simulink model "model"  (R2016a)
(part 3 of 5)

  _CN_258020275_275000_CN_178983951_275000 : powerlib/Elements/Distributed Parameters Line  Phases=3  Frequency=50  Resistance=[0.01273 0.3864]  Inductance="[0.9337e-3  4.1264e-3]"  Capacitance=[12.74e-9 7.751e-9]  Length=72.4946  x1=[8.73114913702011e-11 380000 380000;314.159265358979 314.159265358979 314.159265358979;-0.177670123217348 0.415246442777429 -1.15554988401747]  x2=[1.26090477118469e-09 381852.398472139 381852.398472139;314.159265358979 314.159265358979 314.159265358979;-1.41941675517191 0.415007521738739 -1.15578880505616]  x3=[1.07663708898761e-11 1405.24743813465 1405.24743813466;314.159265358979 314.159265358979 314.159265358979;-2.70558821102223 0.316110507002444 -1.25468581979246]  x4=[8.62234243168895e-12 1405.96374414071 1405.9637441407;314.159265358979 314.159265358979 314.159265358979;0.245769282942371 0.405640215255436 -1.16515611153945]  x5=0.000565541566995742  V1=ones(3,3)  V2=ones(3,3)  I1=ones(3,3)  I2=ones(3,3)  nHarmo=1  Measurements=None
  _CN_258020275_275000_CN_184552955_275000 : powerlib/Elements/Distributed Parameters Line  Phases=3  Frequency=50  Resistance=[0.01273 0.3864]  Inductance="[0.9337e-3  4.1264e-3]"  Capacitance=[12.74e-9 7.751e-9]  Length=80.3266  x1=[8.73114913702011e-11 380000 380000;314.159265358979 314.159265358979 314.159265358979;-0.177670123217348 0.415246442777429 -1.15554988401747]  x2=[1.26090477118469e-09 381852.398472139 381852.398472139;314.159265358979 314.159265358979 314.159265358979;-1.41941675517191 0.415007521738739 -1.15578880505616]  x3=[1.07663708898761e-11 1405.24743813465 1405.24743813466;314.159265358979 314.159265358979 314.159265358979;-2.70558821102223 0.316110507002444 -1.25468581979246]  x4=[8.62234243168895e-12 1405.96374414071 1405.9637441407;314.159265358979 314.159265358979 314.159265358979;0.245769282942371 0.405640215255436 -1.16515611153945]  x5=0.000565541566995742  V1=ones(3,3)  V2=ones(3,3)  I1=ones(3,3)  I2=ones(3,3)  nHarmo=1  Measurements=None
  _CN_262495875_132000_CN_185153858_132000 : powerlib/Elements/Distributed Parameters Line  Phases=3  Frequency=50  Resistance=[0.01273 0.3864]  Inductance="[0.9337e-3  4.1264e-3]"  Capacitance=[12.74e-9 7.751e-9]  Length=25.9236  x1=[8.73114913702011e-11 380000 380000;314.159265358979 314.159265358979 314.159265358979;-0.177670123217348 0.415246442777429 -1.15554988401747]  x2=[1.26090477118469e-09 381852.398472139 381852.398472139;314.159265358979 314.159265358979 314.159265358979;-1.41941675517191 0.415007521738739 -1.15578880505616]  x3=[1.07663708898761e-11 1405.24743813465 1405.24743813466;314.159265358979 314.159265358979 314.159265358979;-2.70558821102223 0.316110507002444 -1.25468581979246]  x4=[8.62234243168895e-12 1405.96374414071 1405.9637441407;314.159265358979 314.159265358979 314.159265358979;0.245769282942371 0.405640215255436 -1.16515611153945]  x5=0.000565541566995742  V1=ones(3,3)  V2=ones(3,3)  I1=ones(3,3)  I2=ones(3,3)  nHarmo=1  Measurements=None
  _CN_28088740_275000_CN_42209860_275000 : powerlib/Elements/Distributed Parameters Line  Phases=3  Frequency=50  Resistance=[0.01273 0.3864]  Inductance="[0.9337e-3  4.1264e-3]"  Capacitance=[12.74e-9 7.751e-9]  Length=14.7594  x1=[8.73114913702011e-11 380000 380000;314.159265358979 314.159265358979 314.159265358979;-0.177670123217348 0.415246442777429 -1.15554988401747]  x2=[1.26090477118469e-09 381852.398472139 381852.398472139;314.159265358979 314.159265358979 314.159265358979;-1.41941675517191 0.415007521738739 -1.15578880505616]  x3=[1.07663708898761e-11 1405.24743813465 1405.24743813466;314.159265358979 314.159265358979 314.159265358979;-2.70558821102223 0.316110507002444 -1.25468581979246]  x4=[8.62234243168895e-12 1405.96374414071 1405.9637441407;314.159265358979 314.159265358979 314.159265358979;0.245769282942371 0.405640215255436 -1.16515611153945]  x5=0.000565541566995742  V1=ones(3,3)  V2=ones(3,3)  I1=ones(3,3)  I2=ones(3,3)  nHarmo=1  Measurements=None
  _CN_28088740_275000_CN_83525879_275000 : powerlib/Elements/Distributed Parameters Line  Phases=3  Frequency=50  Resistance=[0.01273 0.3864]  Inductance="[0.9337e-3  4.1264e-3]"  Capacitance=[12.74e-9 7.751e-9]  Length=33.294  x1=[8.73114913702011e-11 380000 380000;314.159265358979 314.159265358979 314.159265358979;-0.177670123217348 0.415246442777429 -1.15554988401747]  x2=[1.26090477118469e-09 381852.398472139 381852.398472139;314.159265358979 314.159265358979 314.159265358979;-1.41941675517191 0.415007521738739 -1.15578880505616]  x3=[1.07663708898761e-11 1405.24743813465 1405.24743813466;314.159265358979 314.159265358979 314.159265358979;-2.70558821102223 0.316110507002444 -1.25468581979246]  x4=[8.62234243168895e-12 1405.96374414071 1405.9637441407;314.159265358979 314.159265358979 314.159265358979;0.245769282942371 0.405640215255436 -1.16515611153945]  x5=0.000565541566995742  V1=ones(3,3)  V2=ones(3,3)  I1=ones(3,3)  I2=ones(3,3)  nHarmo=1  Measurements=None
  _CN_337464444_132000_CN_337464445_132000 : powerlib/Elements/Distributed Parameters Line  Phases=3  Frequency=50  Resistance=[0.01273 0.3864]  Inductance="[0.9337e-3  4.1264e-3]"  Capacitance=[12.74e-9 7.751e-9]  Length=37.3019  x1=[8.73114913702011e-11 380000 380000;314.159265358979 314.159265358979 314.159265358979;-0.177670123217348 0.415246442777429 -1.15554988401747]  x2=[1.26090477118469e-09 381852.398472139 381852.398472139;314.159265358979 314.159265358979 314.159265358979;-1.41941675517191 0.415007521738739 -1.15578880505616]  x3=[1.07663708898761e-11 1405.24743813465 1405.24743813466;314.159265358979 314.159265358979 314.159265358979;-2.70558821102223 0.316110507002444 -1.25468581979246]  x4=[8.62234243168895e-12 1405.96374414071 1405.9637441407;314.159265358979 314.159265358979 314.159265358979;0.245769282942371 0.405640215255436 -1.16515611153945]  x5=0.000565541566995742  V1=ones(3,3)  V2=ones(3,3)  I1=ones(3,3)  I2=ones(3,3)  nHarmo=1  Measurements=None
  _CN_337464445_132000_CN_120941257_132000 : powerlib/Elements/Distributed Parameters Line  Phases=3  Frequency=50  Resistance=[0.01273 0.3864]  Inductance="[0.9337e-3  4.1264e-3]"  Capacitance=[12.74e-9 7.751e-9]  Length=17.2696  x1=[8.73114913702011e-11 380000 380000;314.159265358979 314.159265358979 314.159265358979;-0.177670123217348 0.415246442777429 -1.15554988401747]  x2=[1.26090477118469e-09 381852.398472139 381852.398472139;314.159265358979 314.159265358979 314.159265358979;-1.41941675517191 0.415007521738739 -1.15578880505616]  x3=[1.07663708898761e-11 1405.24743813465 1405.24743813466;314.159265358979 314.159265358979 314.159265358979;-2.70558821102223 0.316110507002444 -1.25468581979246]  x4=[8.62234243168895e-12 1405.96374414071 1405.9637441407;314.159265358979 314.159265358979 314.159265358979;0.245769282942371 0.405640215255436 -1.16515611153945]  x5=0.000565541566995742  V1=ones(3,3)  V2=ones(3,3)  I1=ones(3,3)  I2=ones(3,3)  nHarmo=1  Measurements=None
  _CN_363326105_275000_CN_179856840_275000 : powerlib/Elements/Distributed Parameters Line  Phases=3  Frequency=50  Resistance=[0.01273 0.3864]  Inductance="[0.9337e-3  4.1264e-3]"  Capacitance=[12.74e-9 7.751e-9]  Length=82.6904  x1=[8.73114913702011e-11 380000 380000;314.159265358979 314.159265358979 314.159265358979;-0.177670123217348 0.415246442777429 -1.15554988401747]  x2=[1.26090477118469e-09 381852.398472139 381852.398472139;314.159265358979 314.159265358979 314.159265358979;-1.41941675517191 0.415007521738739 -1.15578880505616]  x3=[1.07663708898761e-11 1405.24743813465 1405.24743813466;314.159265358979 314.159265358979 314.159265358979;-2.70558821102223 0.316110507002444 -1.25468581979246]  x4=[8.62234243168895e-12 1405.96374414071 1405.9637441407;314.159265358979 314.159265358979 314.159265358979;0.245769282942371 0.405640215255436 -1.16515611153945]  x5=0.000565541566995742  V1=ones(3,3)  V2=ones(3,3)  I1=ones(3,3)  I2=ones(3,3)  nHarmo=1  Measurements=None
  _CN_386388564_400000_CN_418832515_400000 : powerlib/Elements/Distributed Parameters Line  Phases=3  Frequency=50  Resistance=[0.01273 0.3864]  Inductance="[0.9337e-3  4.1264e-3]"  Capacitance=[12.74e-9 7.751e-9]  Length=233.4949  x1=[8.73114913702011e-11 380000 380000;314.159265358979 314.159265358979 314.159265358979;-0.177670123217348 0.415246442777429 -1.15554988401747]  x2=[1.26090477118469e-09 381852.398472139 381852.398472139;314.159265358979 314.159265358979 314.159265358979;-1.41941675517191 0.415007521738739 -1.15578880505616]  x3=[1.07663708898761e-11 1405.24743813465 1405.24743813466;314.159265358979 314.159265358979 314.159265358979;-2.70558821102223 0.316110507002444 -1.25468581979246]  x4=[8.62234243168895e-12 1405.96374414071 1405.9637441407;314.159265358979 314.159265358979 314.159265358979;0.245769282942371 0.405640215255436 -1.16515611153945]  x5=0.000565541566995742  V1=ones(3,3)  V2=ones(3,3)  I1=ones(3,3)  I2=ones(3,3)  nHarmo=1  Measurements=None
  _CN_42209493_132000_CN_81813288_132000 : powerlib/Elements/Distributed Parameters Line  Phases=3  Frequency=50  Resistance=[0.01273 0.3864]  Inductance="[0.9337e-3  4.1264e-3]"  Capacitance=[12.74e-9 7.751e-9]  Length=3.3802  x1=[8.73114913702011e-11 380000 380000;314.159265358979 314.159265358979 314.159265358979;-0.177670123217348 0.415246442777429 -1.15554988401747]  x2=[1.26090477118469e-09 381852.398472139 381852.398472139;314.159265358979 314.159265358979 314.159265358979;-1.41941675517191 0.415007521738739 -1.15578880505616]  x3=[1.07663708898761e-11 1405.24743813465 1405.24743813466;314.159265358979 314.159265358979 314.159265358979;-2.70558821102223 0.316110507002444 -1.25468581979246]  x4=[8.62234243168895e-12 1405.96374414071 1405.9637441407;314.159265358979 314.159265358979 314.159265358979;0.245769282942371 0.405640215255436 -1.16515611153945]  x5=0.000565541566995742  V1=ones(3,3)  V2=ones(3,3)  I1=ones(3,3)  I2=ones(3,3)  nHarmo=1  Measurements=None
  _CN_42209493_275000_CN_81817181_275000 : powerlib/Elements/Distributed Parameters Line  Phases=3  Frequency=50  Resistance=[0.01273 0.3864]  Inductance="[0.9337e-3  4.1264e-3]"  Capacitance=[12.74e-9 7.751e-9]  Length=11.3863  x1=[8.73114913702011e-11 380000 380000;314.159265358979 314.159265358979 314.159265358979;-0.177670123217348 0.415246442777429 -1.15554988401747]  x2=[1.26090477118469e-09 381852.398472139 381852.398472139;314.159265358979 314.159265358979 314.159265358979;-1.41941675517191 0.415007521738739 -1.15578880505616]  x3=[1.07663708898761e-11 1405.24743813465 1405.24743813466;314.159265358979 314.159265358979 314.159265358979;-2.70558821102223 0.316110507002444 -1.25468581979246]  x4=[8.62234243168895e-12 1405.96374414071 1405.9637441407;314.159265358979 314.159265358979 314.159265358979;0.245769282942371 0.405640215255436 -1.16515611153945]  x5=0.000565541566995742  V1=ones(3,3)  V2=ones(3,3)  I1=ones(3,3)  I2=ones(3,3)  nHarmo=1  Measurements=None
  _CN_42209860_275000_CN_178944143_275000 : powerlib/Elements/Distributed Parameters Line  Phases=3  Frequency=50  Resistance=[0.01273 0.3864]  Inductance="[0.9337e-3  4.1264e-3]"  Capacitance=[12.74e-9 7.751e-9]  Length=11.1612  x1=[8.73114913702011e-11 380000 380000;314.159265358979 314.159265358979 314.159265358979;-0.177670123217348 0.415246442777429 -1.15554988401747]  x2=[1.26090477118469e-09 381852.398472139 381852.398472139;314.159265358979 314.159265358979 314.159265358979;-1.41941675517191 0.415007521738739 -1.15578880505616]  x3=[1.07663708898761e-11 1405.24743813465 1405.24743813466;314.159265358979 314.159265358979 314.159265358979;-2.70558821102223 0.316110507002444 -1.25468581979246]  x4=[8.62234243168895e-12 1405.96374414071 1405.9637441407;314.159265358979 314.159265358979 314.159265358979;0.245769282942371 0.405640215255436 -1.16515611153945]  x5=0.000565541566995742  V1=ones(3,3)  V2=ones(3,3)  I1=ones(3,3)  I2=ones(3,3)  nHarmo=1  Measurements=None
  _CN_42209860_275000_CN_42209493_275000 : powerlib/Elements/Distributed Parameters Line  Phases=3  Frequency=50  Resistance=[0.01273 0.3864]  Inductance="[0.9337e-3  4.1264e-3]"  Capacitance=[12.74e-9 7.751e-9]  Length=2.13  x1=[8.73114913702011e-11 380000 380000;314.159265358979 314.159265358979 314.159265358979;-0.177670123217348 0.415246442777429 -1.15554988401747]  x2=[1.26090477118469e-09 381852.398472139 381852.398472139;314.159265358979 314.159265358979 314.159265358979;-1.41941675517191 0.415007521738739 -1.15578880505616]  x3=[1.07663708898761e-11 1405.24743813465 1405.24743813466;314.159265358979 314.159265358979 314.159265358979;-2.70558821102223 0.316110507002444 -1.25468581979246]  x4=[8.62234243168895e-12 1405.96374414071 1405.9637441407;314.159265358979 314.159265358979 314.159265358979;0.245769282942371 0.405640215255436 -1.16515611153945]  x5=0.000565541566995742  V1=ones(3,3)  V2=ones(3,3)  I1=ones(3,3)  I2=ones(3,3)  nHarmo=1  Measurements=None
  _CN_59037450_132000_CN_62191005_132000 : powerlib/Elements/Distributed Parameters Line  Phases=3  Frequency=50  Resistance=[0.01273 0.3864]  Inductance="[0.9337e-3  4.1264e-3]"  Capacitance=[12.74e-9 7.751e-9]  Length=22.8456  x1=[8.73114913702011e-11 380000 380000;314.159265358979 314.159265358979 314.159265358979;-0.177670123217348 0.415246442777429 -1.15554988401747]  x2=[1.26090477118469e-09 381852.398472139 381852.398472139;314.159265358979 314.159265358979 314.159265358979;-1.41941675517191 0.415007521738739 -1.15578880505616]  x3=[1.07663708898761e-11 1405.24743813465 1405.24743813466;314.159265358979 314.159265358979 314.159265358979;-2.70558821102223 0.316110507002444 -1.25468581979246]  x4=[8.62234243168895e-12 1405.96374414071 1405.9637441407;314.159265358979 314.159265358979 314.159265358979;0.245769282942371 0.405640215255436 -1.16515611153945]  x5=0.000565541566995742  V1=ones(3,3)  V2=ones(3,3)  I1=ones(3,3)  I2=ones(3,3)  nHarmo=1  Measurements=None
  _CN_59037450_132000_CN_62208493_132000 : powerlib/Elements/Distributed Parameters Line  Phases=3  Frequency=50  Resistance=[0.01273 0.3864]  Inductance="[0.9337e-3  4.1264e-3]"  Capacitance=[12.74e-9 7.751e-9]  Length=4.1197  x1=[8.73114913702011e-11 380000 380000;314.159265358979 314.159265358979 314.159265358979;-0.177670123217348 0.415246442777429 -1.15554988401747]  x2=[1.26090477118469e-09 381852.398472139 381852.398472139;314.159265358979 314.159265358979 314.159265358979;-1.41941675517191 0.415007521738739 -1.15578880505616]  x3=[1.07663708898761e-11 1405.24743813465 1405.24743813466;314.159265358979 314.159265358979 314.159265358979;-2.70558821102223 0.316110507002444 -1.25468581979246]  x4=[8.62234243168895e-12 1405.96374414071 1405.9637441407;314.159265358979 314.159265358979 314.159265358979;0.245769282942371 0.405640215255436 -1.16515611153945]  x5=0.000565541566995742  V1=ones(3,3)  V2=ones(3,3)  I1=ones(3,3)  I2=ones(3,3)  nHarmo=1  Measurements=None
  _CN_62191005_400000_CN_120584910_400000 : powerlib/Elements/Distributed Parameters Line  Phases=3  Frequency=50  Resistance=[0.01273 0.3864]  Inductance="[0.9337e-3  4.1264e-3]"  Capacitance=[12.74e-9 7.751e-9]  Length=16.2899  x1=[8.73114913702011e-11 380000 380000;314.159265358979 314.159265358979 314.159265358979;-0.177670123217348 0.415246442777429 -1.15554988401747]  x2=[1.26090477118469e-09 381852.398472139 381852.398472139;314.159265358979 314.159265358979 314.159265358979;-1.41941675517191 0.415007521738739 -1.15578880505616]  x3=[1.07663708898761e-11 1405.24743813465 1405.24743813466;314.159265358979 314.159265358979 314.159265358979;-2.70558821102223 0.316110507002444 -1.25468581979246]  x4=[8.62234243168895e-12 1405.96374414071 1405.9637441407;314.159265358979 314.159265358979 314.159265358979;0.245769282942371 0.405640215255436 -1.16515611153945]  x5=0.000565541566995742  V1=ones(3,3)  V2=ones(3,3)  I1=ones(3,3)  I2=ones(3,3)  nHarmo=1  Measurements=None
  _CN_62191005_400000_CN_177800991_400000 : powerlib/Elements/Distributed Parameters Line  Phases=3  Frequency=50  Resistance=[0.01273 0.3864]  Inductance="[0.9337e-3  4.1264e-3]"  Capacitance=[12.74e-9 7.751e-9]  Length=108.9818  x1=[8.73114913702011e-11 380000 380000;314.159265358979 314.159265358979 314.159265358979;-0.177670123217348 0.415246442777429 -1.15554988401747]  x2=[1.26090477118469e-09 381852.398472139 381852.398472139;314.159265358979 314.159265358979 314.159265358979;-1.41941675517191 0.415007521738739 -1.15578880505616]  x3=[1.07663708898761e-11 1405.24743813465 1405.24743813466;314.159265358979 314.159265358979 314.159265358979;-2.70558821102223 0.316110507002444 -1.25468581979246]  x4=[8.62234243168895e-12 1405.96374414071 1405.9637441407;314.159265358979 314.159265358979 314.159265358979;0.245769282942371 0.405640215255436 -1.16515611153945]  x5=0.000565541566995742  V1=ones(3,3)  V2=ones(3,3)  I1=ones(3,3)  I2=ones(3,3)  nHarmo=1  Measurements=None
  _CN_62191005_400000_CN_219384657_400000 : powerlib/Elements/Distributed Parameters Line  Phases=3  Frequency=50  Resistance=[0.01273 0.3864]  Inductance="[0.9337e-3  4.1264e-3]"  Capacitance=[12.74e-9 7.751e-9]  Length=32.1405  x1=[8.73114913702011e-11 380000 380000;314.159265358979 314.159265358979 314.159265358979;-0.177670123217348 0.415246442777429 -1.15554988401747]  x2=[1.26090477118469e-09 381852.398472139 381852.398472139;314.159265358979 314.159265358979 314.159265358979;-1.41941675517191 0.415007521738739 -1.15578880505616]  x3=[1.07663708898761e-11 1405.24743813465 1405.24743813466;314.159265358979 314.159265358979 314.159265358979;-2.70558821102223 0.316110507002444 -1.25468581979246]  x4=[8.62234243168895e-12 1405.96374414071 1405.9637441407;314.159265358979 314.159265358979 314.159265358979;0.245769282942371 0.405640215255436 -1.16515611153945]  x5=0.000565541566995742  V1=ones(3,3)  V2=ones(3,3)  I1=ones(3,3)  I2=ones(3,3)  nHarmo=1  Measurements=None
  _CN_62191005_400000_CN_252396496_132000 : powerlib/Elements/Distributed Parameters Line  Phases=3  Frequency=50  Resistance=[0.01273 0.3864]  Inductance="[0.9337e-3  4.1264e-3]"  Capacitance=[12.74e-9 7.751e-9]  Length=40.4547  x1=[8.73114913702011e-11 380000 380000;314.159265358979 314.159265358979 314.159265358979;-0.177670123217348 0.415246442777429 -1.15554988401747]  x2=[1.26090477118469e-09 381852.398472139 381852.398472139;314.159265358979 314.159265358979 314.159265358979;-1.41941675517191 0.415007521738739 -1.15578880505616]  x3=[1.07663708898761e-11 1405.24743813465 1405.24743813466;314.159265358979 314.159265358979 314.159265358979;-2.70558821102223 0.316110507002444 -1.25468581979246]  x4=[8.62234243168895e-12 1405.96374414071 1405.9637441407;314.159265358979 314.159265358979 314.159265358979;0.245769282942371 0.405640215255436 -1.16515611153945]  x5=0.000565541566995742  V1=ones(3,3)  V2=ones(3,3)  I1=ones(3,3)  I2=ones(3,3)  nHarmo=1  Measurements=None
  _CN_62191005_400000_CN_62193952_400000 : powerlib/Elements/Distributed Parameters Line  Phases=3  Frequency=50  Resistance=[0.01273 0.3864]  Inductance="[0.9337e-3  4.1264e-3]"  Capacitance=[12.74e-9 7.751e-9]  Length=47.199  x1=[8.73114913702011e-11 380000 380000;314.159265358979 314.159265358979 314.159265358979;-0.177670123217348 0.415246442777429 -1.15554988401747]  x2=[1.26090477118469e-09 381852.398472139 381852.398472139;314.159265358979 314.159265358979 314.159265358979;-1.41941675517191 0.415007521738739 -1.15578880505616]  x3=[1.07663708898761e-11 1405.24743813465 1405.24743813466;314.159265358979 314.159265358979 314.159265358979;-2.70558821102223 0.316110507002444 -1.25468581979246]  x4=[8.62234243168895e-12 1405.96374414071 1405.9637441407;314.159265358979 314.159265358979 314.159265358979;0.245769282942371 0.405640215255436 -1.16515611153945]  x5=0.000565541566995742  V1=ones(3,3)  V2=ones(3,3)  I1=ones(3,3)  I2=ones(3,3)  nHarmo=1  Measurements=None
  _CN_62193952_400000_CN_252396496_132000 : powerlib/Elements/Distributed Parameters Line  Phases=3  Frequency=50  Resistance=[0.01273 0.3864]  Inductance="[0.9337e-3  4.1264e-3]"  Capacitance=[12.74e-9 7.751e-9]  Length=31.3538  x1=[8.73114913702011e-11 380000 380000;314.159265358979 314.159265358979 314.159265358979;-0.177670123217348 0.415246442777429 -1.15554988401747]  x2=[1.26090477118469e-09 381852.398472139 381852.398472139;314.159265358979 314.159265358979 314.159265358979;-1.41941675517191 0.415007521738739 -1.15578880505616]  x3=[1.07663708898761e-11 1405.24743813465 1405.24743813466;314.159265358979 314.159265358979 314.159265358979;-2.70558821102223 0.316110507002444 -1.25468581979246]  x4=[8.62234243168895e-12 1405.96374414071 1405.9637441407;314.159265358979 314.159265358979 314.159265358979;0.245769282942371 0.405640215255436 -1.16515611153945]  x5=0.000565541566995742  V1=ones(3,3)  V2=ones(3,3)  I1=ones(3,3)  I2=ones(3,3)  nHarmo=1  Measurements=None
  _CN_62193952_400000_CN_62218063_400000 : powerlib/Elements/Distributed Parameters Line  Phases=3  Frequency=50  Resistance=[0.01273 0.3864]  Inductance="[0.9337e-3  4.1264e-3]"  Capacitance=[12.74e-9 7.751e-9]  Length=12.3981  x1=[8.73114913702011e-11 380000 380000;314.159265358979 314.159265358979 314.159265358979;-0.177670123217348 0.415246442777429 -1.15554988401747]  x2=[1.26090477118469e-09 381852.398472139 381852.398472139;314.159265358979 314.159265358979 314.159265358979;-1.41941675517191 0.415007521738739 -1.15578880505616]  x3=[1.07663708898761e-11 1405.24743813465 1405.24743813466;314.159265358979 314.159265358979 314.159265358979;-2.70558821102223 0.316110507002444 -1.25468581979246]  x4=[8.62234243168895e-12 1405.96374414071 1405.9637441407;314.159265358979 314.159265358979 314.159265358979;0.245769282942371 0.405640215255436 -1.16515611153945]  x5=0.000565541566995742  V1=ones(3,3)  V2=ones(3,3)  I1=ones(3,3)  I2=ones(3,3)  nHarmo=1  Measurements=None
  _CN_62216709_132000_CN_402366747_132000 : powerlib/Elements/Distributed Parameters Line  Phases=3  Frequency=50  Resistance=[0.01273 0.3864]  Inductance="[0.9337e-3  4.1264e-3]"  Capacitance=[12.74e-9 7.751e-9]  Length=1.8763  x1=[8.73114913702011e-11 380000 380000;314.159265358979 314.159265358979 314.159265358979;-0.177670123217348 0.415246442777429 -1.15554988401747]  x2=[1.26090477118469e-09 381852.398472139 381852.398472139;314.159265358979 314.159265358979 314.159265358979;-1.41941675517191 0.415007521738739 -1.15578880505616]  x3=[1.07663708898761e-11 1405.24743813465 1405.24743813466;314.159265358979 314.159265358979 314.159265358979;-2.70558821102223 0.316110507002444 -1.25468581979246]  x4=[8.62234243168895e-12 1405.96374414071 1405.9637441407;314.159265358979 314.159265358979 314.159265358979;0.245769282942371 0.405640215255436 -1.16515611153945]  x5=0.000565541566995742  V1=ones(3,3)  V2=ones(3,3)  I1=ones(3,3)  I2=ones(3,3)  nHarmo=1  Measurements=None
  _CN_62216709_132000_CN_62208493_132000 : powerlib/Elements/Distributed Parameters Line  Phases=3  Frequency=50  Resistance=[0.01273 0.3864]  Inductance="[0.9337e-3  4.1264e-3]"  Capacitance=[12.74e-9 7.751e-9]  Length=6.6911  x1=[8.73114913702011e-11 380000 380000;314.159265358979 314.159265358979 314.159265358979;-0.177670123217348 0.415246442777429 -1.15554988401747]  x2=[1.26090477118469e-09 381852.398472139 381852.398472139;314.159265358979 314.159265358979 314.159265358979;-1.41941675517191 0.415007521738739 -1.15578880505616]  x3=[1.07663708898761e-11 1405.24743813465 1405.24743813466;314.159265358979 314.159265358979 314.159265358979;-2.70558821102223 0.316110507002444 -1.25468581979246]  x4=[8.62234243168895e-12 1405.96374414071 1405.9637441407;314.159265358979 314.159265358979 314.159265358979;0.245769282942371 0.405640215255436 -1.16515611153945]  x5=0.000565541566995742  V1=ones(3,3)  V2=ones(3,3)  I1=ones(3,3)  I2=ones(3,3)  nHarmo=1  Measurements=None
  _CN_62216709_132000_CN_89824175_132000 : powerlib/Elements/Distributed Parameters Line  Phases=3  Frequency=50  Resistance=[0.01273 0.3864]  Inductance="[0.9337e-3  4.1264e-3]"  Capacitance=[12.74e-9 7.751e-9]  Length=9.9569  x1=[8.73114913702011e-11 380000 380000;314.159265358979 314.159265358979 314.159265358979;-0.177670123217348 0.415246442777429 -1.15554988401747]  x2=[1.26090477118469e-09 381852.398472139 381852.398472139;314.159265358979 314.159265358979 314.159265358979;-1.41941675517191 0.415007521738739 -1.15578880505616]  x3=[1.07663708898761e-11 1405.24743813465 1405.24743813466;314.159265358979 314.159265358979 314.159265358979;-2.70558821102223 0.316110507002444 -1.25468581979246]  x4=[8.62234243168895e-12 1405.96374414071 1405.9637441407;314.159265358979 314.159265358979 314.159265358979;0.245769282942371 0.405640215255436 -1.16515611153945]  x5=0.000565541566995742  V1=ones(3,3)  V2=ones(3,3)  I1=ones(3,3)  I2=ones(3,3)  nHarmo=1  Measurements=None
  _CN_62218063_132000_CN_62218065_132000 : powerlib/Elements/Distributed Parameters Line  Phases=3  Frequency=50  Resistance=[0.01273 0.3864]  Inductance="[0.9337e-3  4.1264e-3]"  Capacitance=[12.74e-9 7.751e-9]  Length=4.6832  x1=[8.73114913702011e-11 380000 380000;314.159265358979 314.159265358979 314.159265358979;-0.177670123217348 0.415246442777429 -1.15554988401747]  x2=[1.26090477118469e-09 381852.398472139 381852.398472139;314.159265358979 314.159265358979 314.159265358979;-1.41941675517191 0.415007521738739 -1.15578880505616]  x3=[1.07663708898761e-11 1405.24743813465 1405.24743813466;314.159265358979 314.159265358979 314.159265358979;-2.70558821102223 0.316110507002444 -1.25468581979246]  x4=[8.62234243168895e-12 1405.96374414071 1405.9637441407;314.159265358979 314.159265358979 314.159265358979;0.245769282942371 0.405640215255436 -1.16515611153945]  x5=0.000565541566995742  V1=ones(3,3)  V2=ones(3,3)  I1=ones(3,3)  I2=ones(3,3)  nHarmo=1  Measurements=None
  _CN_62218065_132000_CN_62218069_132000 : powerlib/Elements/Distributed Parameters Line  Phases=3  Frequency=50  Resistance=[0.01273 0.3864]  Inductance="[0.9337e-3  4.1264e-3]"  Capacitance=[12.74e-9 7.751e-9]  Length=3.9185  x1=[8.73114913702011e-11 380000 380000;314.159265358979 314.159265358979 314.159265358979;-0.177670123217348 0.415246442777429 -1.15554988401747]  x2=[1.26090477118469e-09 381852.398472139 381852.398472139;314.159265358979 314.159265358979 314.159265358979;-1.41941675517191 0.415007521738739 -1.15578880505616]  x3=[1.07663708898761e-11 1405.24743813465 1405.24743813466;314.159265358979 314.159265358979 314.159265358979;-2.70558821102223 0.316110507002444 -1.25468581979246]  x4=[8.62234243168895e-12 1405.96374414071 1405.9637441407;314.159265358979 314.159265358979 314.159265358979;0.245769282942371 0.405640215255436 -1.16515611153945]  x5=0.000565541566995742  V1=ones(3,3)  V2=ones(3,3)  I1=ones(3,3)  I2=ones(3,3)  nHarmo=1  Measurements=None
  _CN_62219472_132000_CN_62218063_132000 : powerlib/Elements/Distributed Parameters Line  Phases=3  Frequency=50  Resistance=[0.01273 0.3864]  Inductance="[0.9337e-3  4.1264e-3]"  Capacitance=[12.74e-9 7.751e-9]  Length=7.7115  x1=[8.73114913702011e-11 380000 380000;314.159265358979 314.159265358979 314.159265358979;-0.177670123217348 0.415246442777429 -1.15554988401747]  x2=[1.26090477118469e-09 381852.398472139 381852.398472139;314.159265358979 314.159265358979 314.159265358979;-1.41941675517191 0.415007521738739 -1.15578880505616]  x3=[1.07663708898761e-11 1405.24743813465 1405.24743813466;314.159265358979 314.159265358979 314.159265358979;-2.70558821102223 0.316110507002444 -1.25468581979246]  x4=[8.62234243168895e-12 1405.96374414071 1405.9637441407;314.159265358979 314.159265358979 314.159265358979;0.245769282942371 0.405640215255436 -1.16515611153945]  x5=0.000565541566995742  V1=ones(3,3)  V2=ones(3,3)  I1=ones(3,3)  I2=ones(3,3)  nHarmo=1  Measurements=None
  _CN_65600948_400000_CN_105811523_400000 : powerlib/Elements/Distributed Parameters Line  Phases=3  Frequency=50  Resistance=[0.01273 0.3864]  Inductance="[0.9337e-3  4.1264e-3]"  Capacitance=[12.74e-9 7.751e-9]  Length=143.1893  x1=[8.73114913702011e-11 380000 380000;314.159265358979 314.159265358979 314.159265358979;-0.177670123217348 0.415246442777429 -1.15554988401747]  x2=[1.26090477118469e-09 381852.398472139 381852.398472139;314.159265358979 314.159265358979 314.159265358979;-1.41941675517191 0.415007521738739 -1.15578880505616]  x3=[1.07663708898761e-11 1405.24743813465 1405.24743813466;314.159265358979 314.159265358979 314.159265358979;-2.70558821102223 0.316110507002444 -1.25468581979246]  x4=[8.62234243168895e-12 1405.96374414071 1405.9637441407;314.159265358979 314.159265358979 314.159265358979;0.245769282942371 0.405640215255436 -1.16515611153945]  x5=0.000565541566995742  V1=ones(3,3)  V2=ones(3,3)  I1=ones(3,3)  I2=ones(3,3)  nHarmo=1  Measurements=None
  _CN_65600948_400000_CN_178968761_400000 : powerlib/Elements/Distributed Parameters Line  Phases=3  Frequency=50  Resistance=[0.01273 0.3864]  Inductance="[0.9337e-3  4.1264e-3]"  Capacitance=[12.74e-9 7.751e-9]  Length=54.33  x1=[8.73114913702011e-11 380000 380000;314.159265358979 314.159265358979 314.159265358979;-0.177670123217348 0.415246442777429 -1.15554988401747]  x2=[1.26090477118469e-09 381852.398472139 381852.398472139;314.159265358979 314.159265358979 314.159265358979;-1.41941675517191 0.415007521738739 -1.15578880505616]  x3=[1.07663708898761e-11 1405.24743813465 1405.24743813466;314.159265358979 314.159265358979 314.159265358979;-2.70558821102223 0.316110507002444 -1.25468581979246]  x4=[8.62234243168895e-12 1405.96374414071 1405.9637441407;314.159265358979 314.159265358979 314.159265358979;0.245769282942371 0.405640215255436 -1.16515611153945]  x5=0.000565541566995742  V1=ones(3,3)  V2=ones(3,3)  I1=ones(3,3)  I2=ones(3,3)  nHarmo=1  Measurements=None
  _CN_65600948_400000_CN_185171511_400000 : powerlib/Elements/Distributed Parameters Line  Phases=3  Frequency=50  Resistance=[0.01273 0.3864]  Inductance="[0.9337e-3  4.1264e-3]"  Capacitance=[12.74e-9 7.751e-9]  Length=60.4036  x1=[8.73114913702011e-11 380000 380000;314.159265358979 314.159265358979 314.159265358979;-0.177670123217348 0.415246442777429 -1.15554988401747]  x2=[1.26090477118469e-09 381852.398472139 381852.398472139;314.159265358979 314.159265358979 314.159265358979;-1.41941675517191 0.415007521738739 -1.15578880505616]  x3=[1.07663708898761e-11 1405.24743813465 1405.24743813466;314.159265358979 314.159265358979 314.159265358979;-2.70558821102223 0.316110507002444 -1.25468581979246]  x4=[8.62234243168895e-12 1405.96374414071 1405.9637441407;314.159265358979 314.159265358979 314.159265358979;0.245769282942371 0.405640215255436 -1.16515611153945]  x5=0.000565541566995742  V1=ones(3,3)  V2=ones(3,3)  I1=ones(3,3)  I2=ones(3,3)  nHarmo=1  Measurements=None
  _CN_65600948_400000_CN_418832515_400000 : powerlib/Elements/Distributed Parameters Line  Phases=3  Frequency=50  Resistance=[0.01273 0.3864]  Inductance="[0.9337e-3  4.1264e-3]"  Capacitance=[12.74e-9 7.751e-9]  Length=117.8696  x1=[8.73114913702011e-11 380000 380000;314.159265358979 314.159265358979 314.159265358979;-0.177670123217348 0.415246442777429 -1.15554988401747]  x2=[1.26090477118469e-09 381852.398472139 381852.398472139;314.159265358979 314.159265358979 314.159265358979;-1.41941675517191 0.415007521738739 -1.15578880505616]  x3=[1.07663708898761e-11 1405.24743813465 1405.24743813466;314.159265358979 314.159265358979 314.159265358979;-2.70558821102223 0.316110507002444 -1.25468581979246]  x4=[8.62234243168895e-12 1405.96374414071 1405.9637441407;314.159265358979 314.159265358979 314.159265358979;0.245769282942371 0.405640215255436 -1.16515611153945]  x5=0.000565541566995742  V1=ones(3,3)  V2=ones(3,3)  I1=ones(3,3)  I2=ones(3,3)  nHarmo=1  Measurements=None
  _CN_70586039_132000_CN_84840271_132000 : powerlib/Elements/Distributed Parameters Line  Phases=3  Frequency=50  Resistance=[0.01273 0.3864]  Inductance="[0.9337e-3  4.1264e-3]"  Capacitance=[12.74e-9 7.751e-9]  Length=3.9742  x1=[8.73114913702011e-11 380000 380000;314.159265358979 314.159265358979 314.159265358979;-0.177670123217348 0.415246442777429 -1.15554988401747]  x2=[1.26090477118469e-09 381852.398472139 381852.398472139;314.159265358979 314.159265358979 314.159265358979;-1.41941675517191 0.415007521738739 -1.15578880505616]  x3=[1.07663708898761e-11 1405.24743813465 1405.24743813466;314.159265358979 314.159265358979 314.159265358979;-2.70558821102223 0.316110507002444 -1.25468581979246]  x4=[8.62234243168895e-12 1405.96374414071 1405.9637441407;314.159265358979 314.159265358979 314.159265358979;0.245769282942371 0.405640215255436 -1.16515611153945]  x5=0.000565541566995742  V1=ones(3,3)  V2=ones(3,3)  I1=ones(3,3)  I2=ones(3,3)  nHarmo=1  Measurements=None
  _CN_75136015_275000_CN_178950118_275000 : powerlib/Elements/Distributed Parameters Line  Phases=3  Frequency=50  Resistance=[0.01273 0.3864]  Inductance="[0.9337e-3  4.1264e-3]"  Capacitance=[12.74e-9 7.751e-9]  Length=25.9057  x1=[8.73114913702011e-11 380000 380000;314.159265358979 314.159265358979 314.159265358979;-0.177670123217348 0.415246442777429 -1.15554988401747]  x2=[1.26090477118469e-09 381852.398472139 381852.398472139;314.159265358979 314.159265358979 314.159265358979;-1.41941675517191 0.415007521738739 -1.15578880505616]  x3=[1.07663708898761e-11 1405.24743813465 1405.24743813466;314.159265358979 314.159265358979 314.159265358979;-2.70558821102223 0.316110507002444 -1.25468581979246]  x4=[8.62234243168895e-12 1405.96374414071 1405.9637441407;314.159265358979 314.159265358979 314.159265358979;0.245769282942371 0.405640215255436 -1.16515611153945]  x5=0.000565541566995742  V1=ones(3,3)  V2=ones(3,3)  I1=ones(3,3)  I2=ones(3,3)  nHarmo=1  Measurements=None
  _CN_75136015_275000_CN_187432497_275000 : powerlib/Elements/Distributed Parameters Line  Phases=3  Frequency=50  Resistance=[0.01273 0.3864]  Inductance="[0.9337e-3  4.1264e-3]"  Capacitance=[12.74e-9 7.751e-9]  Length=22.212  x1=[8.73114913702011e-11 380000 380000;314.159265358979 314.159265358979 314.159265358979;-0.177670123217348 0.415246442777429 -1.15554988401747]  x2=[1.26090477118469e-09 381852.398472139 381852.398472139;314.159265358979 314.159265358979 314.159265358979;-1.41941675517191 0.415007521738739 -1.15578880505616]  x3=[1.07663708898761e-11 1405.24743813465 1405.24743813466;314.159265358979 314.159265358979 314.159265358979;-2.70558821102223 0.316110507002444 -1.25468581979246]  x4=[8.62234243168895e-12 1405.96374414071 1405.9637441407;314.159265358979 314.159265358979 314.159265358979;0.245769282942371 0.405640215255436 -1.16515611153945]  x5=0.000565541566995742  V1=ones(3,3)  V2=ones(3,3)  I1=ones(3,3)  I2=ones(3,3)  nHarmo=1  Measurements=None
  _CN_75136015_275000_CN_32509808_275000 : powerlib/Elements/Distributed Parameters Line  Phases=3  Frequency=50  Resistance=[0.01273 0.3864]  Inductance="[0.9337e-3  4.1264e-3]"  Capacitance=[12.74e-9 7.751e-9]  Length=26.4297  x1=[8.73114913702011e-11 380000 380000;314.159265358979 314.159265358979 314.159265358979;-0.177670123217348 0.415246442777429 -1.15554988401747]  x2=[1.26090477118469e-09 381852.398472139 381852.398472139;314.159265358979 314.159265358979 314.159265358979;-1.41941675517191 0.415007521738739 -1.15578880505616]  x3=[1.07663708898761e-11 1405.24743813465 1405.24743813466;314.159265358979 314.159265358979 314.159265358979;-2.70558821102223 0.316110507002444 -1.25468581979246]  x4=[8.62234243168895e-12 1405.96374414071 1405.9637441407;314.159265358979 314.159265358979 314.159265358979;0.245769282942371 0.405640215255436 -1.16515611153945]  x5=0.000565541566995742  V1=ones(3,3)  V2=ones(3,3)  I1=ones(3,3)  I2=ones(3,3)  nHarmo=1  Measurements=None
  _CN_75136015_275000_CN_84197405_275000 : powerlib/Elements/Distributed Parameters Line  Phases=3  Frequency=50  Resistance=[0.01273 0.3864]  Inductance="[0.9337e-3  4.1264e-3]"  Capacitance=[12.74e-9 7.751e-9]  Length=19.738  x1=[8.73114913702011e-11 380000 380000;314.159265358979 314.159265358979 314.159265358979;-0.177670123217348 0.415246442777429 -1.15554988401747]  x2=[1.26090477118469e-09 381852.398472139 381852.398472139;314.159265358979 314.159265358979 314.159265358979;-1.41941675517191 0.415007521738739 -1.15578880505616]  x3=[1.07663708898761e-11 1405.24743813465 1405.24743813466;314.159265358979 314.159265358979 314.159265358979;-2.70558821102223 0.316110507002444 -1.25468581979246]  x4=[8.62234243168895e-12 1405.96374414071 1405.9637441407;314.159265358979 314.159265358979 314.159265358979;0.245769282942371 0.405640215255436 -1.16515611153945]  x5=0.000565541566995742  V1=ones(3,3)  V2=ones(3,3)  I1=ones(3,3)  I2=ones(3,3)  nHarmo=1  Measurements=None
  _CN_75136015_400000_CN_83525879_400000 : powerlib/Elements/Distributed Parameters Line  Phases=3  Frequency=50  Resistance=[0.01273 0.3864]  Inductance="[0.9337e-3  4.1264e-3]"  Capacitance=[12.74e-9 7.751e-9]  Length=22.498  x1=[8.73114913702011e-11 380000 380000;314.159265358979 314.159265358979 314.159265358979;-0.177670123217348 0.415246442777429 -1.15554988401747]  x2=[1.26090477118469e-09 381852.398472139 381852.398472139;314.159265358979 314.159265358979 314.159265358979;-1.41941675517191 0.415007521738739 -1.15578880505616]  x3=[1.07663708898761e-11 1405.24743813465 1405.24743813466;314.159265358979 314.159265358979 314.159265358979;-2.70558821102223 0.316110507002444 -1.25468581979246]  x4=[8.62234243168895e-12 1405.96374414071 1405.9637441407;314.159265358979 314.159265358979 314.159265358979;0.245769282942371 0.405640215255436 -1.16515611153945]  x5=0.000565541566995742  V1=ones(3,3)  V2=ones(3,3)  I1=ones(3,3)  I2=ones(3,3)  nHarmo=1  Measurements=None
  _CN_75136015_400000_CN_87404898_400000 : powerlib/Elements/Distributed Parameters Line  Phases=3  Frequency=50  Resistance=[0.01273 0.3864]  Inductance="[0.9337e-3  4.1264e-3]"  Capacitance=[12.74e-9 7.751e-9]  Length=78.9956  x1=[8.73114913702011e-11 380000 380000;314.159265358979 314.159265358979 314.159265358979;-0.177670123217348 0.415246442777429 -1.15554988401747]  x2=[1.26090477118469e-09 381852.398472139 381852.398472139;314.159265358979 314.159265358979 314.159265358979;-1.41941675517191 0.415007521738739 -1.15578880505616]  x3=[1.07663708898761e-11 1405.24743813465 1405.24743813466;314.159265358979 314.159265358979 314.159265358979;-2.70558821102223 0.316110507002444 -1.25468581979246]  x4=[8.62234243168895e-12 1405.96374414071 1405.9637441407;314.159265358979 314.159265358979 314.159265358979;0.245769282942371 0.405640215255436 -1.16515611153945]  x5=0.000565541566995742  V1=ones(3,3)  V2=ones(3,3)  I1=ones(3,3)  I2=ones(3,3)  nHarmo=1  Measurements=None
  _CN_82014905_275000_CN_81817181_275000 : powerlib/Elements/Distributed Parameters Line  Phases=3  Frequency=50  Resistance=[0.01273 0.3864]  Inductance="[0.9337e-3  4.1264e-3]"  Capacitance=[12.74e-9 7.751e-9]  Length=33.2026  x1=[8.73114913702011e-11 380000 380000;314.159265358979 314.159265358979 314.159265358979;-0.177670123217348 0.415246442777429 -1.15554988401747]  x2=[1.26090477118469e-09 381852.398472139 381852.398472139;314.159265358979 314.159265358979 314.159265358979;-1.41941675517191 0.415007521738739 -1.15578880505616]  x3=[1.07663708898761e-11 1405.24743813465 1405.24743813466;314.159265358979 314.159265358979 314.159265358979;-2.70558821102223 0.316110507002444 -1.25468581979246]  x4=[8.62234243168895e-12 1405.96374414071 1405.9637441407;314.159265358979 314.159265358979 314.159265358979;0.245769282942371 0.405640215255436 -1.16515611153945]  x5=0.000565541566995742  V1=ones(3,3)  V2=ones(3,3)  I1=ones(3,3)  I2=ones(3,3)  nHarmo=1  Measurements=None
  _CN_82014905_275000_CN_83188568_275000 : powerlib/Elements/Distributed Parameters Line  Phases=3  Frequency=50  Resistance=[0.01273 0.3864]  Inductance="[0.9337e-3  4.1264e-3]"  Capacitance=[12.74e-9 7.751e-9]  Length=18.7293  x1=[8.73114913702011e-11 380000 380000;314.159265358979 314.159265358979 314.159265358979;-0.177670123217348 0.415246442777429 -1.15554988401747]  x2=[1.26090477118469e-09 381852.398472139 381852.398472139;314.159265358979 314.159265358979 314.159265358979;-1.41941675517191 0.415007521738739 -1.15578880505616]  x3=[1.07663708898761e-11 1405.24743813465 1405.24743813466;314.159265358979 314.159265358979 314.159265358979;-2.70558821102223 0.316110507002444 -1.25468581979246]  x4=[8.62234243168895e-12 1405.96374414071 1405.9637441407;314.159265358979 314.159265358979 314.159265358979;0.245769282942371 0.405640215255436 -1.16515611153945]  x5=0.000565541566995742  V1=ones(3,3)  V2=ones(3,3)  I1=ones(3,3)  I2=ones(3,3)  nHarmo=1  Measurements=None
  _CN_83188525_132000_CN_83244979_132000 : powerlib/Elements/Distributed Parameters Line  Phases=3  Frequency=50  Resistance=[0.01273 0.3864]  Inductance="[0.9337e-3  4.1264e-3]"  Capacitance=[12.74e-9 7.751e-9]  Length=4.671  x1=[8.73114913702011e-11 380000 380000;314.159265358979 314.159265358979 314.159265358979;-0.177670123217348 0.415246442777429 -1.15554988401747]  x2=[1.26090477118469e-09 381852.398472139 381852.398472139;314.159265358979 314.159265358979 314.159265358979;-1.41941675517191 0.415007521738739 -1.15578880505616]  x3=[1.07663708898761e-11 1405.24743813465 1405.24743813466;314.159265358979 314.159265358979 314.159265358979;-2.70558821102223 0.316110507002444 -1.25468581979246]  x4=[8.62234243168895e-12 1405.96374414071 1405.9637441407;314.159265358979 314.159265358979 314.159265358979;0.245769282942371 0.405640215255436 -1.16515611153945]  x5=0.000565541566995742  V1=ones(3,3)  V2=ones(3,3)  I1=ones(3,3)  I2=ones(3,3)  nHarmo=1  Measurements=None
  _CN_83188568_132000_CN_83244979_132000 : powerlib/Elements/Distributed Parameters Line  Phases=3  Frequency=50  Resistance=[0.01273 0.3864]  Inductance="[0.9337e-3  4.1264e-3]"  Capacitance=[12.74e-9 7.751e-9]  Length=10.0814  x1=[8.73114913702011e-11 380000 380000;314.159265358979 314.159265358979 314.159265358979;-0.177670123217348 0.415246442777429 -1.15554988401747]  x2=[1.26090477118469e-09 381852.398472139 381852.398472139;314.159265358979 314.159265358979 314.159265358979;-1.41941675517191 0.415007521738739 -1.15578880505616]  x3=[1.07663708898761e-11 1405.24743813465 1405.24743813466;314.159265358979 314.159265358979 314.159265358979;-2.70558821102223 0.316110507002444 -1.25468581979246]  x4=[8.62234243168895e-12 1405.96374414071 1405.9637441407;314.159265358979 314.159265358979 314.159265358979;0.245769282942371 0.405640215255436 -1.16515611153945]  x5=0.000565541566995742  V1=ones(3,3)  V2=ones(3,3)  I1=ones(3,3)  I2=ones(3,3)  nHarmo=1  Measurements=None
  _CN_83525876_275000_CN_83525879_275000 : powerlib/Elements/Distributed Parameters Line  Phases=3  Frequency=50  Resistance=[0.01273 0.3864]  Inductance="[0.9337e-3  4.1264e-3]"  Capacitance=[12.74e-9 7.751e-9]  Length=5.2794  x1=[8.73114913702011e-11 380000 380000;314.159265358979 314.159265358979 314.159265358979;-0.177670123217348 0.415246442777429 -1.15554988401747]  x2=[1.26090477118469e-09 381852.398472139 381852.398472139;314.159265358979 314.159265358979 314.159265358979;-1.41941675517191 0.415007521738739 -1.15578880505616]  x3=[1.07663708898761e-11 1405.24743813465 1405.24743813466;314.159265358979 314.159265358979 314.159265358979;-2.70558821102223 0.316110507002444 -1.25468581979246]  x4=[8.62234243168895e-12 1405.96374414071 1405.9637441407;314.159265358979 314.159265358979 314.159265358979;0.245769282942371 0.405640215255436 -1.16515611153945]  x5=0.000565541566995742  V1=ones(3,3)  V2=ones(3,3)  I1=ones(3,3)  I2=ones(3,3)  nHarmo=1  Measurements=None
  _CN_83888980_275000_CN_83188568_275000 : powerlib/Elements/Distributed Parameters Line  Phases=3  Frequency=50  Resistance=[0.01273 0.3864]  Inductance="[0.9337e-3  4.1264e-3]"  Capacitance=[12.74e-9 7.751e-9]  Length=13.0673  x1=[8.73114913702011e-11 380000 380000;314.159265358979 314.159265358979 314.159265358979;-0.177670123217348 0.415246442777429 -1.15554988401747]  x2=[1.26090477118469e-09 381852.398472139 381852.398472139;314.159265358979 314.159265358979 314.159265358979;-1.41941675517191 0.415007521738739 -1.15578880505616]  x3=[1.07663708898761e-11 1405.24743813465 1405.24743813466;314.159265358979 314.159265358979 314.159265358979;-2.70558821102223 0.316110507002444 -1.25468581979246]  x4=[8.62234243168895e-12 1405.96374414071 1405.9637441407;314.159265358979 314.159265358979 314.159265358979;0.245769282942371 0.405640215255436 -1.16515611153945]  x5=0.000565541566995742  V1=ones(3,3)  V2=ones(3,3)  I1=ones(3,3)  I2=ones(3,3)  nHarmo=1  Measurements=None
  _CN_83888980_275000_CN_83945972_275000 : powerlib/Elements/Distributed Parameters Line  Phases=3  Frequency=50  Resistance=[0.01273 0.3864]  Inductance="[0.9337e-3  4.1264e-3]"  Capacitance=[12.74e-9 7.751e-9]  Length=11.4186  x1=[8.73114913702011e-11 380000 380000;314.159265358979 314.159265358979 314.159265358979;-0.177670123217348 0.415246442777429 -1.15554988401747]  x2=[1.26090477118469e-09 381852.398472139 381852.398472139;314.159265358979 314.159265358979 314.159265358979;-1.41941675517191 0.415007521738739 -1.15578880505616]  x3=[1.07663708898761e-11 1405.24743813465 1405.24743813466;314.159265358979 314.159265358979 314.159265358979;-2.70558821102223 0.316110507002444 -1.25468581979246]  x4=[8.62234243168895e-12 1405.96374414071 1405.9637441407;314.159265358979 314.159265358979 314.159265358979;0.245769282942371 0.405640215255436 -1.16515611153945]  x5=0.000565541566995742  V1=ones(3,3)  V2=ones(3,3)  I1=ones(3,3)  I2=ones(3,3)  nHarmo=1  Measurements=None
  _CN_83950316_275000_CN_418842091_275000 : powerlib/Elements/Distributed Parameters Line  Phases=3  Frequency=50  Resistance=[0.01273 0.3864]  Inductance="[0.9337e-3  4.1264e-3]"  Capacitance=[12.74e-9 7.751e-9]  Length=101.1996  x1=[8.73114913702011e-11 380000 380000;314.159265358979 314.159265358979 314.159265358979;-0.177670123217348 0.415246442777429 -1.15554988401747]  x2=[1.26090477118469e-09 381852.398472139 381852.398472139;314.159265358979 314.159265358979 314.159265358979;-1.41941675517191 0.415007521738739 -1.15578880505616]  x3=[1.07663708898761e-11 1405.24743813465 1405.24743813466;314.159265358979 314.159265358979 314.159265358979;-2.70558821102223 0.316110507002444 -1.25468581979246]  x4=[8.62234243168895e-12 1405.96374414071 1405.9637441407;314.159265358979 314.159265358979 314.159265358979;0.245769282942371 0.405640215255436 -1.16515611153945]  x5=0.000565541566995742  V1=ones(3,3)  V2=ones(3,3)  I1=ones(3,3)  I2=ones(3,3)  nHarmo=1  Measurements=None
  _CN_83951788_132000_CN_83537732_132000 : powerlib/Elements/Distributed Parameters Line  Phases=3  Frequency=50  Resistance=[0.01273 0.3864]  Inductance="[0.9337e-3  4.1264e-3]"  Capacitance=[12.74e-9 7.751e-9]  Length=48.6352  x1=[8.73114913702011e-11 380000 380000;314.159265358979 314.159265358979 314.159265358979;-0.177670123217348 0.415246442777429 -1.15554988401747]  x2=[1.26090477118469e-09 381852.398472139 381852.398472139;314.159265358979 314.159265358979 314.159265358979;-1.41941675517191 0.415007521738739 -1.15578880505616]  x3=[1.07663708898761e-11 1405.24743813465 1405.24743813466;314.159265358979 314.159265358979 314.159265358979;-2.70558821102223 0.316110507002444 -1.25468581979246]  x4=[8.62234243168895e-12 1405.96374414071 1405.9637441407;314.159265358979 314.159265358979 314.159265358979;0.245769282942371 0.405640215255436 -1.16515611153945]  x5=0.000565541566995742  V1=ones(3,3)  V2=ones(3,3)  I1=ones(3,3)  I2=ones(3,3)  nHarmo=1  Measurements=None
  _CN_83951788_275000_CN_178983951_275000 : powerlib/Elements/Distributed Parameters Line  Phases=3  Frequency=50  Resistance=[0.01273 0.3864]  Inductance="[0.9337e-3  4.1264e-3]"  Capacitance=[12.74e-9 7.751e-9]  Length=100.2508  x1=[8.73114913702011e-11 380000 380000;314.159265358979 314.159265358979 314.159265358979;-0.177670123217348 0.415246442777429 -1.15554988401747]  x2=[1.26090477118469e-09 381852.398472139 381852.398472139;314.159265358979 314.159265358979 314.159265358979;-1.41941675517191 0.415007521738739 -1.15578880505616]  x3=[1.07663708898761e-11 1405.24743813465 1405.24743813466;314.159265358979 314.159265358979 314.159265358979;-2.70558821102223 0.316110507002444 -1.25468581979246]  x4=[8.62234243168895e-12 1405.96374414071 1405.9637441407;314.159265358979 314.159265358979 314.159265358979;0.245769282942371 0.405640215255436 -1.16515611153945]  x5=0.000565541566995742  V1=ones(3,3)  V2=ones(3,3)  I1=ones(3,3)  I2=ones(3,3)  nHarmo=1  Measurements=None
  _CN_83951788_275000_CN_83525879_275000 : powerlib/Elements/Distributed Parameters Line  Phases=3  Frequency=50  Resistance=[0.01273 0.3864]  Inductance="[0.9337e-3  4.1264e-3]"  Capacitance=[12.74e-9 7.751e-9]  Length=11.3634  x1=[8.73114913702011e-11 380000 380000;314.159265358979 314.159265358979 314.159265358979;-0.177670123217348 0.415246442777429 -1.15554988401747]  x2=[1.26090477118469e-09 381852.398472139 381852.398472139;314.159265358979 314.159265358979 314.159265358979;-1.41941675517191 0.415007521738739 -1.15578880505616]  x3=[1.07663708898761e-11 1405.24743813465 1405.24743813466;314.159265358979 314.159265358979 314.159265358979;-2.70558821102223 0.316110507002444 -1.25468581979246]  x4=[8.62234243168895e-12 1405.96374414071 1405.9637441407;314.159265358979 314.159265358979 314.159265358979;0.245769282942371 0.405640215255436 -1.16515611153945]  x5=0.000565541566995742  V1=ones(3,3)  V2=ones(3,3)  I1=ones(3,3)  I2=ones(3,3)  nHarmo=1  Measurements=None
  _CN_84197284_132000_CN_84840271_132000 : powerlib/Elements/Distributed Parameters Line  Phases=3  Frequency=50  Resistance=[0.01273 0.3864]  Inductance="[0.9337e-3  4.1264e-3]"  Capacitance=[12.74e-9 7.751e-9]  Length=8.4586  x1=[8.73114913702011e-11 380000 380000;314.159265358979 314.159265358979 314.159265358979;-0.177670123217348 0.415246442777429 -1.15554988401747]  x2=[1.26090477118469e-09 381852.398472139 381852.398472139;314.159265358979 314.159265358979 314.159265358979;-1.41941675517191 0.415007521738739 -1.15578880505616]  x3=[1.07663708898761e-11 1405.24743813465 1405.24743813466;314.159265358979 314.159265358979 314.159265358979;-2.70558821102223 0.316110507002444 -1.25468581979246]  x4=[8.62234243168895e-12 1405.96374414071 1405.9637441407;314.159265358979 314.159265358979 314.159265358979;0.245769282942371 0.405640215255436 -1.16515611153945]  x5=0.000565541566995742  V1=ones(3,3)  V2=ones(3,3)  I1=ones(3,3)  I2=ones(3,3)  nHarmo=1  Measurements=None
  _CN_84197405_132000_CN_418863865_132000 : powerlib/Elements/Distributed Parameters Line  Phases=3  Frequency=50  Resistance=[0.01273 0.3864]  Inductance="[0.9337e-3  4.1264e-3]"  Capacitance=[12.74e-9 7.751e-9]  Length=4.9598  x1=[8.73114913702011e-11 380000 380000;314.159265358979 314.159265358979 314.159265358979;-0.177670123217348 0.415246442777429 -1.15554988401747]  x2=[1.26090477118469e-09 381852.398472139 381852.398472139;314.159265358979 314.159265358979 314.159265358979;-1.41941675517191 0.415007521738739 -1.15578880505616]  x3=[1.07663708898761e-11 1405.24743813465 1405.24743813466;314.159265358979 314.159265358979 314.159265358979;-2.70558821102223 0.316110507002444 -1.25468581979246]  x4=[8.62234243168895e-12 1405.96374414071 1405.9637441407;314.159265358979 314.159265358979 314.159265358979;0.245769282942371 0.405640215255436 -1.16515611153945]  x5=0.000565541566995742  V1=ones(3,3)  V2=ones(3,3)  I1=ones(3,3)  I2=ones(3,3)  nHarmo=1  Measurements=None
  _CN_84197405_132000_CN_84197350_132000 : powerlib/Elements/Distributed Parameters Line  Phases=3  Frequency=50  Resistance=[0.01273 0.3864]  Inductance="[0.9337e-3  4.1264e-3]"  Capacitance=[12.74e-9 7.751e-9]  Length=5.5168  x1=[8.73114913702011e-11 380000 380000;314.159265358979 314.159265358979 314.159265358979;-0.177670123217348 0.415246442777429 -1.15554988401747]  x2=[1.26090477118469e-09 381852.398472139 381852.398472139;314.159265358979 314.159265358979 314.159265358979;-1.41941675517191 0.415007521738739 -1.15578880505616]  x3=[1.07663708898761e-11 1405.24743813465 1405.24743813466;314.159265358979 314.159265358979 314.159265358979;-2.70558821102223 0.316110507002444 -1.25468581979246]  x4=[8.62234243168895e-12 1405.96374414071 1405.9637441407;314.159265358979 314.159265358979 314.159265358979;0.245769282942371 0.405640215255436 -1.16515611153945]  x5=0.000565541566995742  V1=ones(3,3)  V2=ones(3,3)  I1=ones(3,3)  I2=ones(3,3)  nHarmo=1  Measurements=None
  _CN_84198429_132000_CN_84198438_132000 : powerlib/Elements/Distributed Parameters Line  Phases=3  Frequency=50  Resistance=[0.01273 0.3864]  Inductance="[0.9337e-3  4.1264e-3]"  Capacitance=[12.74e-9 7.751e-9]  Length=5.3821  x1=[8.73114913702011e-11 380000 380000;314.159265358979 314.159265358979 314.159265358979;-0.177670123217348 0.415246442777429 -1.15554988401747]  x2=[1.26090477118469e-09 381852.398472139 381852.398472139;314.159265358979 314.159265358979 314.159265358979;-1.41941675517191 0.415007521738739 -1.15578880505616]  x3=[1.07663708898761e-11 1405.24743813465 1405.24743813466;314.159265358979 314.159265358979 314.159265358979;-2.70558821102223 0.316110507002444 -1.25468581979246]  x4=[8.62234243168895e-12 1405.96374414071 1405.9637441407;314.159265358979 314.159265358979 314.159265358979;0.245769282942371 0.405640215255436 -1.16515611153945]  x5=0.000565541566995742  V1=ones(3,3)  V2=ones(3,3)  I1=ones(3,3)  I2=ones(3,3)  nHarmo=1  Measurements=None
  _CN_84198429_132000_CN_84273857_132000 : powerlib/Elements/Distributed Parameters Line  Phases=3  Frequency=50  Resistance=[0.01273 0.3864]  Inductance="[0.9337e-3  4.1264e-3]"  Capacitance=[12.74e-9 7.751e-9]  Length=4.5482  x1=[8.73114913702011e-11 380000 380000;314.159265358979 314.159265358979 314.159265358979;-0.177670123217348 0.415246442777429 -1.15554988401747]  x2=[1.26090477118469e-09 381852.398472139 381852.398472139;314.159265358979 314.159265358979 314.159265358979;-1.41941675517191 0.415007521738739 -1.15578880505616]  x3=[1.07663708898761e-11 1405.24743813465 1405.24743813466;314.159265358979 314.159265358979 314.159265358979;-2.70558821102223 0.316110507002444 -1.25468581979246]  x4=[8.62234243168895e-12 1405.96374414071 1405.9637441407;314.159265358979 314.159265358979 314.159265358979;0.245769282942371 0.405640215255436 -1.16515611153945]  x5=0.000565541566995742  V1=ones(3,3)  V2=ones(3,3)  I1=ones(3,3)  I2=ones(3,3)  nHarmo=1  Measurements=None
  _CN_84198444_132000_CN_84197405_132000 : powerlib/Elements/Distributed Parameters Line  Phases=3  Frequency=50  Resistance=[0.01273 0.3864]  Inductance="[0.9337e-3  4.1264e-3]"  Capacitance=[12.74e-9 7.751e-9]  Length=1.6958  x1=[8.73114913702011e-11 380000 380000;314.159265358979 314.159265358979 314.159265358979;-0.177670123217348 0.415246442777429 -1.15554988401747]  x2=[1.26090477118469e-09 381852.398472139 381852.398472139;314.159265358979 314.159265358979 314.159265358979;-1.41941675517191 0.415007521738739 -1.15578880505616]  x3=[1.07663708898761e-11 1405.24743813465 1405.24743813466;314.159265358979 314.159265358979 314.159265358979;-2.70558821102223 0.316110507002444 -1.25468581979246]  x4=[8.62234243168895e-12 1405.96374414071 1405.9637441407;314.159265358979 314.159265358979 314.159265358979;0.245769282942371 0.405640215255436 -1.16515611153945]  x5=0.000565541566995742  V1=ones(3,3)  V2=ones(3,3)  I1=ones(3,3)  I2=ones(3,3)  nHarmo=1  Measurements=None
  _CN_84198444_132000_CN_84273857_132000 : powerlib/Elements/Distributed Parameters Line  Phases=3  Frequency=50  Resistance=[0.01273 0.3864]  Inductance="[0.9337e-3  4.1264e-3]"  Capacitance=[12.74e-9 7.751e-9]  Length=16.872  x1=[8.73114913702011e-11 380000 380000;314.159265358979 314.159265358979 314.159265358979;-0.177670123217348 0.415246442777429 -1.15554988401747]  x2=[1.26090477118469e-09 381852.398472139 381852.398472139;314.159265358979 314.159265358979 314.159265358979;-1.41941675517191 0.415007521738739 -1.15578880505616]  x3=[1.07663708898761e-11 1405.24743813465 1405.24743813466;314.159265358979 314.159265358979 314.159265358979;-2.70558821102223 0.316110507002444 -1.25468581979246]  x4=[8.62234243168895e-12 1405.96374414071 1405.9637441407;314.159265358979 314.159265358979 314.159265358979;0.245769282942371 0.405640215255436 -1.16515611153945]  x5=0.000565541566995742  V1=ones(3,3)  V2=ones(3,3)  I1=ones(3,3)  I2=ones(3,3)  nHarmo=1  Measurements=None
  _CN_84273851_132000_CN_84273857_132000 : powerlib/Elements/Distributed Parameters Line  Phases=3  Frequency=50  Resistance=[0.01273 0.3864]  Inductance="[0.9337e-3  4.1264e-3]"  Capacitance=[12.74e-9 7.751e-9]  Length=2.7108  x1=[8.73114913702011e-11 380000 380000;314.159265358979 314.159265358979 314.159265358979;-0.177670123217348 0.415246442777429 -1.15554988401747]  x2=[1.26090477118469e-09 381852.398472139 381852.398472139;314.159265358979 314.159265358979 314.159265358979;-1.41941675517191 0.415007521738739 -1.15578880505616]  x3=[1.07663708898761e-11 1405.24743813465 1405.24743813466;314.159265358979 314.159265358979 314.159265358979;-2.70558821102223 0.316110507002444 -1.25468581979246]  x4=[8.62234243168895e-12 1405.96374414071 1405.9637441407;314.159265358979 314.159265358979 314.159265358979;0.245769282942371 0.405640215255436 -1.16515611153945]  x5=0.000565541566995742  V1=ones(3,3)  V2=ones(3,3)  I1=ones(3,3)  I2=ones(3,3)  nHarmo=1  Measurements=None
  _CN_84273851_132000_CN_84274096_132000 : powerlib/Elements/Distributed Parameters Line  Phases=3  Frequency=50  Resistance=[0.01273 0.3864]  Inductance="[0.9337e-3  4.1264e-3]"  Capacitance=[12.74e-9 7.751e-9]  Length=8.3143  x1=[8.73114913702011e-11 380000 380000;314.159265358979 314.159265358979 314.159265358979;-0.177670123217348 0.415246442777429 -1.15554988401747]  x2=[1.26090477118469e-09 381852.398472139 381852.398472139;314.159265358979 314.159265358979 314.159265358979;-1.41941675517191 0.415007521738739 -1.15578880505616]  x3=[1.07663708898761e-11 1405.24743813465 1405.24743813466;314.159265358979 314.159265358979 314.159265358979;-2.70558821102223 0.316110507002444 -1.25468581979246]  x4=[8.62234243168895e-12 1405.96374414071 1405.9637441407;314.159265358979 314.159265358979 314.159265358979;0.245769282942371 0.405640215255436 -1.16515611153945]  x5=0.000565541566995742  V1=ones(3,3)  V2=ones(3,3)  I1=ones(3,3)  I2=ones(3,3)  nHarmo=1  Measurements=None
  _CN_84273857_132000_CN_84273858_132000 : powerlib/Elements/Distributed Parameters Line  Phases=3  Frequency=50  Resistance=[0.01273 0.3864]  Inductance="[0.9337e-3  4.1264e-3]"  Capacitance=[12.74e-9 7.751e-9]  Length=0.12997  x1=[8.73114913702011e-11 380000 380000;314.159265358979 314.159265358979 314.159265358979;-0.177670123217348 0.415246442777429 -1.15554988401747]  x2=[1.26090477118469e-09 381852.398472139 381852.398472139;314.159265358979 314.159265358979 314.159265358979;-1.41941675517191 0.415007521738739 -1.15578880505616]  x3=[1.07663708898761e-11 1405.24743813465 1405.24743813466;314.159265358979 314.159265358979 314.159265358979;-2.70558821102223 0.316110507002444 -1.25468581979246]  x4=[8.62234243168895e-12 1405.96374414071 1405.9637441407;314.159265358979 314.159265358979 314.159265358979;0.245769282942371 0.405640215255436 -1.16515611153945]  x5=0.000565541566995742  V1=ones(3,3)  V2=ones(3,3)  I1=ones(3,3)  I2=ones(3,3)  nHarmo=1  Measurements=None
  _CN_84274092_132000_CN_84274096_132000 : powerlib/Elements/Distributed Parameters Line  Phases=3  Frequency=50  Resistance=[0.01273 0.3864]  Inductance="[0.9337e-3  4.1264e-3]"  Capacitance=[12.74e-9 7.751e-9]  Length=5.0115  x1=[8.73114913702011e-11 380000 380000;314.159265358979 314.159265358979 314.159265358979;-0.177670123217348 0.415246442777429 -1.15554988401747]  x2=[1.26090477118469e-09 381852.398472139 381852.398472139;314.159265358979 314.159265358979 314.159265358979;-1.41941675517191 0.415007521738739 -1.15578880505616]  x3=[1.07663708898761e-11 1405.24743813465 1405.24743813466;314.159265358979 314.159265358979 314.159265358979;-2.70558821102223 0.316110507002444 -1.25468581979246]  x4=[8.62234243168895e-12 1405.96374414071 1405.9637441407;314.159265358979 314.159265358979 314.159265358979;0.245769282942371 0.405640215255436 -1.16515611153945]  x5=0.000565541566995742  V1=ones(3,3)  V2=ones(3,3)  I1=ones(3,3)  I2=ones(3,3)  nHarmo=1  Measurements=None
  _CN_84274092_275000_CN_83525879_275000 : powerlib/Elements/Distributed Parameters Line  Phases=3  Frequency=50  Resistance=[0.01273 0.3864]  Inductance="[0.9337e-3  4.1264e-3]"  Capacitance=[12.74e-9 7.751e-9]  Length=10.2554  x1=[8.73114913702011e-11 380000 380000;314.159265358979 314.159265358979 314.159265358979;-0.177670123217348 0.415246442777429 -1.15554988401747]  x2=[1.26090477118469e-09 381852.398472139 381852.398472139;314.159265358979 314.159265358979 314.159265358979;-1.41941675517191 0.415007521738739 -1.15578880505616]  x3=[1.07663708898761e-11 1405.24743813465 1405.24743813466;314.159265358979 314.159265358979 314.159265358979;-2.70558821102223 0.316110507002444 -1.25468581979246]  x4=[8.62234243168895e-12 1405.96374414071 1405.9637441407;314.159265358979 314.159265358979 314.159265358979;0.245769282942371 0.405640215255436 -1.16515611153945]  x5=0.000565541566995742  V1=ones(3,3)  V2=ones(3,3)  I1=ones(3,3)  I2=ones(3,3)  nHarmo=1  Measurements=None
  _CN_84360372_132000_CN_84274092_132000 : powerlib/Elements/Distributed Parameters Line  Phases=3  Frequency=50  Resistance=[0.01273 0.3864]  Inductance="[0.9337e-3  4.1264e-3]"  Capacitance=[12.74e-9 7.751e-9]  Length=9.2342  x1=[8.73114913702011e-11 380000 380000;314.159265358979 314.159265358979 314.159265358979;-0.177670123217348 0.415246442777429 -1.15554988401747]  x2=[1.26090477118469e-09 381852.398472139 381852.398472139;314.159265358979 314.159265358979 314.159265358979;-1.41941675517191 0.415007521738739 -1.15578880505616]  x3=[1.07663708898761e-11 1405.24743813465 1405.24743813466;314.159265358979 314.159265358979 314.159265358979;-2.70558821102223 0.316110507002444 -1.25468581979246]  x4=[8.62234243168895e-12 1405.96374414071 1405.9637441407;314.159265358979 314.159265358979 314.159265358979;0.245769282942371 0.405640215255436 -1.16515611153945]  x5=0.000565541566995742  V1=ones(3,3)  V2=ones(3,3)  I1=ones(3,3)  I2=ones(3,3)  nHarmo=1  Measurements=None
  _CN_84391364_275000_CN_136695854_275000 : powerlib/Elements/Distributed Parameters Line  Phases=3  Frequency=50  Resistance=[0.01273 0.3864]  Inductance="[0.9337e-3  4.1264e-3]"  Capacitance=[12.74e-9 7.751e-9]  Length=58.5968  x1=[8.73114913702011e-11 380000 380000;314.159265358979 314.159265358979 314.159265358979;-0.177670123217348 0.415246442777429 -1.15554988401747]  x2=[1.26090477118469e-09 381852.398472139 381852.398472139;314.159265358979 314.159265358979 314.159265358979;-1.41941675517191 0.415007521738739 -1.15578880505616]  x3=[1.07663708898761e-11 1405.24743813465 1405.24743813466;314.159265358979 314.159265358979 314.159265358979;-2.70558821102223 0.316110507002444 -1.25468581979246]  x4=[8.62234243168895e-12 1405.96374414071 1405.9637441407;314.159265358979 314.159265358979 314.159265358979;0.245769282942371 0.405640215255436 -1.16515611153945]  x5=0.000565541566995742  V1=ones(3,3)  V2=ones(3,3)  I1=ones(3,3)  I2=ones(3,3)  nHarmo=1  Measurements=None
  _CN_84391364_275000_CN_136695855_275000 : powerlib/Elements/Distributed Parameters Line  Phases=3  Frequency=50  Resistance=[0.01273 0.3864]  Inductance="[0.9337e-3  4.1264e-3]"  Capacitance=[12.74e-9 7.751e-9]  Length=17.4531  x1=[8.73114913702011e-11 380000 380000;314.159265358979 314.159265358979 314.159265358979;-0.177670123217348 0.415246442777429 -1.15554988401747]  x2=[1.26090477118469e-09 381852.398472139 381852.398472139;314.159265358979 314.159265358979 314.159265358979;-1.41941675517191 0.415007521738739 -1.15578880505616]  x3=[1.07663708898761e-11 1405.24743813465 1405.24743813466;314.159265358979 314.159265358979 314.159265358979;-2.70558821102223 0.316110507002444 -1.25468581979246]  x4=[8.62234243168895e-12 1405.96374414071 1405.9637441407;314.159265358979 314.159265358979 314.159265358979;0.245769282942371 0.405640215255436 -1.16515611153945]  x5=0.000565541566995742  V1=ones(3,3)  V2=ones(3,3)  I1=ones(3,3)  I2=ones(3,3)  nHarmo=1  Measurements=None
  _CN_84391364_275000_CN_418842091_275000 : powerlib/Elements/Distributed Parameters Line  Phases=3  Frequency=50  Resistance=[0.01273 0.3864]  Inductance="[0.9337e-3  4.1264e-3]"  Capacitance=[12.74e-9 7.751e-9]  Length=66.6943  x1=[8.73114913702011e-11 380000 380000;314.159265358979 314.159265358979 314.159265358979;-0.177670123217348 0.415246442777429 -1.15554988401747]  x2=[1.26090477118469e-09 381852.398472139 381852.398472139;314.159265358979 314.159265358979 314.159265358979;-1.41941675517191 0.415007521738739 -1.15578880505616]  x3=[1.07663708898761e-11 1405.24743813465 1405.24743813466;314.159265358979 314.159265358979 314.159265358979;-2.70558821102223 0.316110507002444 -1.25468581979246]  x4=[8.62234243168895e-12 1405.96374414071 1405.9637441407;314.159265358979 314.159265358979 314.159265358979;0.245769282942371 0.405640215255436 -1.16515611153945]  x5=0.000565541566995742  V1=ones(3,3)  V2=ones(3,3)  I1=ones(3,3)  I2=ones(3,3)  nHarmo=1  Measurements=None
  _CN_84569471_132000_CN_84569484_132000 : powerlib/Elements/Distributed Parameters Line  Phases=3  Frequency=50  Resistance=[0.01273 0.3864]  Inductance="[0.9337e-3  4.1264e-3]"  Capacitance=[12.74e-9 7.751e-9]  Length=8.8879  x1=[8.73114913702011e-11 380000 380000;314.159265358979 314.159265358979 314.159265358979;-0.177670123217348 0.415246442777429 -1.15554988401747]  x2=[1.26090477118469e-09 381852.398472139 381852.398472139;314.159265358979 314.159265358979 314.159265358979;-1.41941675517191 0.415007521738739 -1.15578880505616]  x3=[1.07663708898761e-11 1405.24743813465 1405.24743813466;314.159265358979 314.159265358979 314.159265358979;-2.70558821102223 0.316110507002444 -1.25468581979246]  x4=[8.62234243168895e-12 1405.96374414071 1405.9637441407;314.159265358979 314.159265358979 314.159265358979;0.245769282942371 0.405640215255436 -1.16515611153945]  x5=0.000565541566995742  V1=ones(3,3)  V2=ones(3,3)  I1=ones(3,3)  I2=ones(3,3)  nHarmo=1  Measurements=None
  _CN_84569471_132000_CN_84569494_132000 : powerlib/Elements/Distributed Parameters Line  Phases=3  Frequency=50  Resistance=[0.01273 0.3864]  Inductance="[0.9337e-3  4.1264e-3]"  Capacitance=[12.74e-9 7.751e-9]  Length=6.7619  x1=[8.73114913702011e-11 380000 380000;314.159265358979 314.159265358979 314.159265358979;-0.177670123217348 0.415246442777429 -1.15554988401747]  x2=[1.26090477118469e-09 381852.398472139 381852.398472139;314.159265358979 314.159265358979 314.159265358979;-1.41941675517191 0.415007521738739 -1.15578880505616]  x3=[1.07663708898761e-11 1405.24743813465 1405.24743813466;314.159265358979 314.159265358979 314.159265358979;-2.70558821102223 0.316110507002444 -1.25468581979246]  x4=[8.62234243168895e-12 1405.96374414071 1405.9637441407;314.159265358979 314.159265358979 314.159265358979;0.245769282942371 0.405640215255436 -1.16515611153945]  x5=0.000565541566995742  V1=ones(3,3)  V2=ones(3,3)  I1=ones(3,3)  I2=ones(3,3)  nHarmo=1  Measurements=None
  _CN_84569484_132000_CN_84571572_132000 : powerlib/Elements/Distributed Parameters Line  Phases=3  Frequency=50  Resistance=[0.01273 0.3864]  Inductance="[0.9337e-3  4.1264e-3]"  Capacitance=[12.74e-9 7.751e-9]  Length=6.0944  x1=[8.73114913702011e-11 380000 380000;314.159265358979 314.159265358979 314.159265358979;-0.177670123217348 0.415246442777429 -1.15554988401747]  x2=[1.26090477118469e-09 381852.398472139 381852.398472139;314.159265358979 314.159265358979 314.159265358979;-1.41941675517191 0.415007521738739 -1.15578880505616]  x3=[1.07663708898761e-11 1405.24743813465 1405.24743813466;314.159265358979 314.159265358979 314.159265358979;-2.70558821102223 0.316110507002444 -1.25468581979246]  x4=[8.62234243168895e-12 1405.96374414071 1405.9637441407;314.159265358979 314.159265358979 314.159265358979;0.245769282942371 0.405640215255436 -1.16515611153945]  x5=0.000565541566995742  V1=ones(3,3)  V2=ones(3,3)  I1=ones(3,3)  I2=ones(3,3)  nHarmo=1  Measurements=None
  _CN_84569494_132000_CN_84274092_132000 : powerlib/Elements/Distributed Parameters Line  Phases=3  Frequency=50  Resistance=[0.01273 0.3864]  Inductance="[0.9337e-3  4.1264e-3]"  Capacitance=[12.74e-9 7.751e-9]  Length=4.5408  x1=[8.73114913702011e-11 380000 380000;314.159265358979 314.159265358979 314.159265358979;-0.177670123217348 0.415246442777429 -1.15554988401747]  x2=[1.26090477118469e-09 381852.398472139 381852.398472139;314.159265358979 314.159265358979 314.159265358979;-1.41941675517191 0.415007521738739 -1.15578880505616]  x3=[1.07663708898761e-11 1405.24743813465 1405.24743813466;314.159265358979 314.159265358979 314.159265358979;-2.70558821102223 0.316110507002444 -1.25468581979246]  x4=[8.62234243168895e-12 1405.96374414071 1405.9637441407;314.159265358979 314.159265358979 314.159265358979;0.245769282942371 0.405640215255436 -1.16515611153945]  x5=0.000565541566995742  V1=ones(3,3)  V2=ones(3,3)  I1=ones(3,3)  I2=ones(3,3)  nHarmo=1  Measurements=None
  _CN_84830388_132000_CN_84830394_132000 : powerlib/Elements/Distributed Parameters Line  Phases=3  Frequency=50  Resistance=[0.01273 0.3864]  Inductance="[0.9337e-3  4.1264e-3]"  Capacitance=[12.74e-9 7.751e-9]  Length=7.3782  x1=[8.73114913702011e-11 380000 380000;314.159265358979 314.159265358979 314.159265358979;-0.177670123217348 0.415246442777429 -1.15554988401747]  x2=[1.26090477118469e-09 381852.398472139 381852.398472139;314.159265358979 314.159265358979 314.159265358979;-1.41941675517191 0.415007521738739 -1.15578880505616]  x3=[1.07663708898761e-11 1405.24743813465 1405.24743813466;314.159265358979 314.159265358979 314.159265358979;-2.70558821102223 0.316110507002444 -1.25468581979246]  x4=[8.62234243168895e-12 1405.96374414071 1405.9637441407;314.159265358979 314.159265358979 314.159265358979;0.245769282942371 0.405640215255436 -1.16515611153945]  x5=0.000565541566995742  V1=ones(3,3)  V2=ones(3,3)  I1=ones(3,3)  I2=ones(3,3)  nHarmo=1  Measurements=None
  _CN_87434264_400000_CN_167540668_400000 : powerlib/Elements/Distributed Parameters Line  Phases=3  Frequency=50  Resistance=[0.01273 0.3864]  Inductance="[0.9337e-3  4.1264e-3]"  Capacitance=[12.74e-9 7.751e-9]  Length=108.92  x1=[8.73114913702011e-11 380000 380000;314.159265358979 314.159265358979 314.159265358979;-0.177670123217348 0.415246442777429 -1.15554988401747]  x2=[1.26090477118469e-09 381852.398472139 381852.398472139;314.159265358979 314.159265358979 314.159265358979;-1.41941675517191 0.415007521738739 -1.15578880505616]  x3=[1.07663708898761e-11 1405.24743813465 1405.24743813466;314.159265358979 314.159265358979 314.159265358979;-2.70558821102223 0.316110507002444 -1.25468581979246]  x4=[8.62234243168895e-12 1405.96374414071 1405.9637441407;314.159265358979 314.159265358979 314.159265358979;0.245769282942371 0.405640215255436 -1.16515611153945]  x5=0.000565541566995742  V1=ones(3,3)  V2=ones(3,3)  I1=ones(3,3)  I2=ones(3,3)  nHarmo=1  Measurements=None
  _CN_87434264_400000_CN_178240542_400000 : powerlib/Elements/Distributed Parameters Line  Phases=3  Frequency=50  Resistance=[0.01273 0.3864]  Inductance="[0.9337e-3  4.1264e-3]"  Capacitance=[12.74e-9 7.751e-9]  Length=16.6544  x1=[8.73114913702011e-11 380000 380000;314.159265358979 314.159265358979 314.159265358979;-0.177670123217348 0.415246442777429 -1.15554988401747]  x2=[1.26090477118469e-09 381852.398472139 381852.398472139;314.159265358979 314.159265358979 314.159265358979;-1.41941675517191 0.415007521738739 -1.15578880505616]  x3=[1.07663708898761e-11 1405.24743813465 1405.24743813466;314.159265358979 314.159265358979 314.159265358979;-2.70558821102223 0.316110507002444 -1.25468581979246]  x4=[8.62234243168895e-12 1405.96374414071 1405.9637441407;314.159265358979 314.159265358979 314.159265358979;0.245769282942371 0.405640215255436 -1.16515611153945]  x5=0.000565541566995742  V1=ones(3,3)  V2=ones(3,3)  I1=ones(3,3)  I2=ones(3,3)  nHarmo=1  Measurements=None
  _CN_87434264_400000_CN_182408147_400000 : powerlib/Elements/Distributed Parameters Line  Phases=3  Frequency=50  Resistance=[0.01273 0.3864]  Inductance="[0.9337e-3  4.1264e-3]"  Capacitance=[12.74e-9 7.751e-9]  Length=204.1851  x1=[8.73114913702011e-11 380000 380000;314.159265358979 314.159265358979 314.159265358979;-0.177670123217348 0.415246442777429 -1.15554988401747]  x2=[1.26090477118469e-09 381852.398472139 381852.398472139;314.159265358979 314.159265358979 314.159265358979;-1.41941675517191 0.415007521738739 -1.15578880505616]  x3=[1.07663708898761e-11 1405.24743813465 1405.24743813466;314.159265358979 314.159265358979 314.159265358979;-2.70558821102223 0.316110507002444 -1.25468581979246]  x4=[8.62234243168895e-12 1405.96374414071 1405.9637441407;314.159265358979 314.159265358979 314.159265358979;0.245769282942371 0.405640215255436 -1.16515611153945]  x5=0.000565541566995742  V1=ones(3,3)  V2=ones(3,3)  I1=ones(3,3)  I2=ones(3,3)  nHarmo=1  Measurements=None
  _CN_87434264_400000_CN_184201271_400000 : powerlib/Elements/Distributed Parameters Line  Phases=3  Frequency=50  Resistance=[0.01273 0.3864]  Inductance="[0.9337e-3  4.1264e-3]"  Capacitance=[12.74e-9 7.751e-9]  Length=100.1591  x1=[8.73114913702011e-11 380000 380000;314.159265358979 314.159265358979 314.159265358979;-0.177670123217348 0.415246442777429 -1.15554988401747]  x2=[1.26090477118469e-09 381852.398472139 381852.398472139;314.159265358979 314.159265358979 314.159265358979;-1.41941675517191 0.415007521738739 -1.15578880505616]  x3=[1.07663708898761e-11 1405.24743813465 1405.24743813466;314.159265358979 314.159265358979 314.159265358979;-2.70558821102223 0.316110507002444 -1.25468581979246]  x4=[8.62234243168895e-12 1405.96374414071 1405.9637441407;314.159265358979 314.159265358979 314.159265358979;0.245769282942371 0.405640215255436 -1.16515611153945]  x5=0.000565541566995742  V1=ones(3,3)  V2=ones(3,3)  I1=ones(3,3)  I2=ones(3,3)  nHarmo=1  Measurements=None
  _CN_87434264_400000_CN_87404898_400000 : powerlib/Elements/Distributed Parameters Line  Phases=3  Frequency=50  Resistance=[0.01273 0.3864]  Inductance="[0.9337e-3  4.1264e-3]"  Capacitance=[12.74e-9 7.751e-9]  Length=23.0501  x1=[8.73114913702011e-11 380000 380000;314.159265358979 314.159265358979 314.159265358979;-0.177670123217348 0.415246442777429 -1.15554988401747]  x2=[1.26090477118469e-09 381852.398472139 381852.398472139;314.159265358979 314.159265358979 314.159265358979;-1.41941675517191 0.415007521738739 -1.15578880505616]  x3=[1.07663708898761e-11 1405.24743813465 1405.24743813466;314.159265358979 314.159265358979 314.159265358979;-2.70558821102223 0.316110507002444 -1.25468581979246]  x4=[8.62234243168895e-12 1405.96374414071 1405.9637441407;314.159265358979 314.159265358979 314.159265358979;0.245769282942371 0.405640215255436 -1.16515611153945]  x5=0.000565541566995742  V1=ones(3,3)  V2=ones(3,3)  I1=ones(3,3)  I2=ones(3,3)  nHarmo=1  Measurements=None
  _CN_89173873_400000_CN_142414070_400000 : powerlib/Elements/Distributed Parameters Line  Phases=3  Frequency=50  Resistance=[0.01273 0.3864]  Inductance="[0.9337e-3  4.1264e-3]"  Capacitance=[12.74e-9 7.751e-9]  Length=102.59  x1=[8.73114913702011e-11 380000 380000;314.159265358979 314.159265358979 314.159265358979;-0.177670123217348 0.415246442777429 -1.15554988401747]  x2=[1.26090477118469e-09 381852.398472139 381852.398472139;314.159265358979 314.159265358979 314.159265358979;-1.41941675517191 0.415007521738739 -1.15578880505616]  x3=[1.07663708898761e-11 1405.24743813465 1405.24743813466;314.159265358979 314.159265358979 314.159265358979;-2.70558821102223 0.316110507002444 -1.25468581979246]  x4=[8.62234243168895e-12 1405.96374414071 1405.9637441407;314.159265358979 314.159265358979 314.159265358979;0.245769282942371 0.405640215255436 -1.16515611153945]  x5=0.000565541566995742  V1=ones(3,3)  V2=ones(3,3)  I1=ones(3,3)  I2=ones(3,3)  nHarmo=1  Measurements=None
  _CN_89824175_132000_CN_189101371_132000 : powerlib/Elements/Distributed Parameters Line  Phases=3  Frequency=50  Resistance=[0.01273 0.3864]  Inductance="[0.9337e-3  4.1264e-3]"  Capacitance=[12.74e-9 7.751e-9]  Length=3.3072  x1=[8.73114913702011e-11 380000 380000;314.159265358979 314.159265358979 314.159265358979;-0.177670123217348 0.415246442777429 -1.15554988401747]  x2=[1.26090477118469e-09 381852.398472139 381852.398472139;314.159265358979 314.159265358979 314.159265358979;-1.41941675517191 0.415007521738739 -1.15578880505616]  x3=[1.07663708898761e-11 1405.24743813465 1405.24743813466;314.159265358979 314.159265358979 314.159265358979;-2.70558821102223 0.316110507002444 -1.25468581979246]  x4=[8.62234243168895e-12 1405.96374414071 1405.9637441407;314.159265358979 314.159265358979 314.159265358979;0.245769282942371 0.405640215255436 -1.16515611153945]  x5=0.000565541566995742  V1=ones(3,3)  V2=ones(3,3)  I1=ones(3,3)  I2=ones(3,3)  nHarmo=1  Measurements=None
  _CN_89830761_132000_CN_62191005_132000 : powerlib/Elements/Distributed Parameters Line  Phases=3  Frequency=50  Resistance=[0.01273 0.3864]  Inductance="[0.9337e-3  4.1264e-3]"  Capacitance=[12.74e-9 7.751e-9]  Length=15.5009  x1=[8.73114913702011e-11 380000 380000;314.159265358979 314.159265358979 314.159265358979;-0.177670123217348 0.415246442777429 -1.15554988401747]  x2=[1.26090477118469e-09 381852.398472139 381852.398472139;314.159265358979 314.159265358979 314.159265358979;-1.41941675517191 0.415007521738739 -1.15578880505616]  x3=[1.07663708898761e-11 1405.24743813465 1405.24743813466;314.159265358979 314.159265358979 314.159265358979;-2.70558821102223 0.316110507002444 -1.25468581979246]  x4=[8.62234243168895e-12 1405.96374414071 1405.9637441407;314.159265358979 314.159265358979 314.159265358979;0.245769282942371 0.405640215255436 -1.16515611153945]  x5=0.000565541566995742  V1=ones(3,3)  V2=ones(3,3)  I1=ones(3,3)  I2=ones(3,3)  nHarmo=1  Measurements=None
  _CN_90454383_400000_CN_89637370_400000 : powerlib/Elements/Distributed Parameters Line  Phases=3  Frequency=50  Resistance=[0.01273 0.3864]  Inductance="[0.9337e-3  4.1264e-3]"  Capacitance=[12.74e-9 7.751e-9]  Length=107.5633  x1=[8.73114913702011e-11 380000 380000;314.159265358979 314.159265358979 314.159265358979;-0.177670123217348 0.415246442777429 -1.15554988401747]  x2=[1.26090477118469e-09 381852.398472139 381852.398472139;314.159265358979 314.159265358979 314.159265358979;-1.41941675517191 0.415007521738739 -1.15578880505616]  x3=[1.07663708898761e-11 1405.24743813465 1405.24743813466;314.159265358979 314.159265358979 314.159265358979;-2.70558821102223 0.316110507002444 -1.25468581979246]  x4=[8.62234243168895e-12 1405.96374414071 1405.9637441407;314.159265358979 314.159265358979 314.159265358979;0.245769282942371 0.405640215255436 -1.16515611153945]  x5=0.000565541566995742  V1=ones(3,3)  V2=ones(3,3)  I1=ones(3,3)  I2=ones(3,3)  nHarmo=1  Measurements=None
  _CN_91979987_132000_CN_103754184_132000 : powerlib/Elements/Distributed Parameters Line  Phases=3  Frequency=50  Resistance=[0.01273 0.3864]  Inductance="[0.9337e-3  4.1264e-3]"  Capacitance=[12.74e-9 7.751e-9]  Length=1.9674  x1=[8.73114913702011e-11 380000 380000;314.159265358979 314.159265358979 314.159265358979;-0.177670123217348 0.415246442777429 -1.15554988401747]  x2=[1.26090477118469e-09 381852.398472139 381852.398472139;314.159265358979 314.159265358979 314.159265358979;-1.41941675517191 0.415007521738739 -1.15578880505616]  x3=[1.07663708898761e-11 1405.24743813465 1405.24743813466;314.159265358979 314.159265358979 314.159265358979;-2.70558821102223 0.316110507002444 -1.25468581979246]  x4=[8.62234243168895e-12 1405.96374414071 1405.9637441407;314.159265358979 314.159265358979 314.159265358979;0.245769282942371 0.405640215255436 -1.16515611153945]  x5=0.000565541566995742  V1=ones(3,3)  V2=ones(3,3)  I1=ones(3,3)  I2=ones(3,3)  nHarmo=1  Measurements=None
  _CN_91979994_132000_CN_171699035_132000 : powerlib/Elements/Distributed Parameters Line  Phases=3  Frequency=50  Resistance=[0.01273 0.3864]  Inductance="[0.9337e-3  4.1264e-3]"  Capacitance=[12.74e-9 7.751e-9]  Length=143.7962  x1=[8.73114913702011e-11 380000 380000;314.159265358979 314.159265358979 314.159265358979;-0.177670123217348 0.415246442777429 -1.15554988401747]  x2=[1.26090477118469e-09 381852.398472139 381852.398472139;314.159265358979 314.159265358979 314.159265358979;-1.41941675517191 0.415007521738739 -1.15578880505616]  x3=[1.07663708898761e-11 1405.24743813465 1405.24743813466;314.159265358979 314.159265358979 314.159265358979;-2.70558821102223 0.316110507002444 -1.25468581979246]  x4=[8.62234243168895e-12 1405.96374414071 1405.9637441407;314.159265358979 314.159265358979 314.159265358979;0.245769282942371 0.405640215255436 -1.16515611153945]  x5=0.000565541566995742  V1=ones(3,3)  V2=ones(3,3)  I1=ones(3,3)  I2=ones(3,3)  nHarmo=1  Measurements=None
  _CN_91979995_132000_CN_169667549_132000 : powerlib/Elements/Distributed Parameters Line  Phases=3  Frequency=50  Resistance=[0.01273 0.3864]  Inductance="[0.9337e-3  4.1264e-3]"  Capacitance=[12.74e-9 7.751e-9]  Length=11.9745  x1=[8.73114913702011e-11 380000 380000;314.159265358979 314.159265358979 314.159265358979;-0.177670123217348 0.415246442777429 -1.15554988401747]  x2=[1.26090477118469e-09 381852.398472139 381852.398472139;314.159265358979 314.159265358979 314.159265358979;-1.41941675517191 0.415007521738739 -1.15578880505616]  x3=[1.07663708898761e-11 1405.24743813465 1405.24743813466;314.159265358979 314.159265358979 314.159265358979;-2.70558821102223 0.316110507002444 -1.25468581979246]  x4=[8.62234243168895e-12 1405.96374414071 1405.9637441407;314.159265358979 314.159265358979 314.159265358979;0.245769282942371 0.405640215255436 -1.16515611153945]  x5=0.000565541566995742  V1=ones(3,3)  V2=ones(3,3)  I1=ones(3,3)  I2=ones(3,3)  nHarmo=1  Measurements=None
  _CN_92343043_275000_CN_191269219_275000 : powerlib/Elements/Distributed Parameters Line  Phases=3  Frequency=50  Resistance=[0.01273 0.3864]  Inductance="[0.9337e-3  4.1264e-3]"  Capacitance=[12.74e-9 7.751e-9]  Length=46.2025  x1=[8.73114913702011e-11 380000 380000;314.159265358979 314.159265358979 314.159265358979;-0.177670123217348 0.415246442777429 -1.15554988401747]  x2=[1.26090477118469e-09 381852.398472139 381852.398472139;314.159265358979 314.159265358979 314.159265358979;-1.41941675517191 0.415007521738739 -1.15578880505616]  x3=[1.07663708898761e-11 1405.24743813465 1405.24743813466;314.159265358979 314.159265358979 314.159265358979;-2.70558821102223 0.316110507002444 -1.25468581979246]  x4=[8.62234243168895e-12 1405.96374414071 1405.9637441407;314.159265358979 314.159265358979 314.159265358979;0.245769282942371 0.405640215255436 -1.16515611153945]  x5=0.000565541566995742  V1=ones(3,3)  V2=ones(3,3)  I1=ones(3,3)  I2=ones(3,3)  nHarmo=1  Measurements=None
  _CN_92348290_275000_CN_217505021_275000 : powerlib/Elements/Distributed Parameters Line  Phases=3  Frequency=50  Resistance=[0.01273 0.3864]  Inductance="[0.9337e-3  4.1264e-3]"  Capacitance=[12.74e-9 7.751e-9]  Length=68.2308  x1=[8.73114913702011e-11 380000 380000;314.159265358979 314.159265358979 314.159265358979;-0.177670123217348 0.415246442777429 -1.15554988401747]  x2=[1.26090477118469e-09 381852.398472139 381852.398472139;314.159265358979 314.159265358979 314.159265358979;-1.41941675517191 0.415007521738739 -1.15578880505616]  x3=[1.07663708898761e-11 1405.24743813465 1405.24743813466;314.159265358979 314.159265358979 314.159265358979;-2.70558821102223 0.316110507002444 -1.25468581979246]  x4=[8.62234243168895e-12 1405.96374414071 1405.9637441407;314.159265358979 314.159265358979 314.159265358979;0.245769282942371 0.405640215255436 -1.16515611153945]  x5=0.000565541566995742  V1=ones(3,3)  V2=ones(3,3)  I1=ones(3,3)  I2=ones(3,3)  nHarmo=1  Measurements=None
  _CN_92348290_400000_CN_142414070_400000 : powerlib/Elements/Distributed Parameters Line  Phases=3  Frequency=50  Resistance=[0.01273 0.3864]  Inductance="[0.9337e-3  4.1264e-3]"  Capacitance=[12.74e-9 7.751e-9]  Length=216.178  x1=[8.73114913702011e-11 380000 380000;314.159265358979 314.159265358979 314.159265358979;-0.177670123217348 0.415246442777429 -1.15554988401747]  x2=[1.26090477118469e-09 381852.398472139 381852.398472139;314.159265358979 314.159265358979 314.159265358979;-1.41941675517191 0.415007521738739 -1.15578880505616]  x3=[1.07663708898761e-11 1405.24743813465 1405.24743813466;314.159265358979 314.159265358979 314.159265358979;-2.70558821102223 0.316110507002444 -1.25468581979246]  x4=[8.62234243168895e-12 1405.96374414071 1405.9637441407;314.159265358979 314.159265358979 314.159265358979;0.245769282942371 0.405640215255436 -1.16515611153945]  x5=0.000565541566995742  V1=ones(3,3)  V2=ones(3,3)  I1=ones(3,3)  I2=ones(3,3)  nHarmo=1  Measurements=None
  _CN_92348290_400000_CN_181366662_400000 : powerlib/Elements/Distributed Parameters Line  Phases=3  Frequency=50  Resistance=[0.01273 0.3864]  Inductance="[0.9337e-3  4.1264e-3]"  Capacitance=[12.74e-9 7.751e-9]  Length=13.5405  x1=[8.73114913702011e-11 380000 380000;314.159265358979 314.159265358979 314.159265358979;-0.177670123217348 0.415246442777429 -1.15554988401747]  x2=[1.26090477118469e-09 381852.398472139 381852.398472139;314.159265358979 314.159265358979 314.159265358979;-1.41941675517191 0.415007521738739 -1.15578880505616]  x3=[1.07663708898761e-11 1405.24743813465 1405.24743813466;314.159265358979 314.159265358979 314.159265358979;-2.70558821102223 0.316110507002444 -1.25468581979246]  x4=[8.62234243168895e-12 1405.96374414071 1405.9637441407;314.159265358979 314.159265358979 314.159265358979;0.245769282942371 0.405640215255436 -1.16515611153945]  x5=0.000565541566995742  V1=ones(3,3)  V2=ones(3,3)  I1=ones(3,3)  I2=ones(3,3)  nHarmo=1  Measurements=None
  _CN_92348290_400000_CN_386388564_400000 : powerlib/Elements/Distributed Parameters Line  Phases=3  Frequency=50  Resistance=[0.01273 0.3864]  Inductance="[0.9337e-3  4.1264e-3]"  Capacitance=[12.74e-9 7.751e-9]  Length=137.994  x1=[8.73114913702011e-11 380000 380000;314.159265358979 314.159265358979 314.159265358979;-0.177670123217348 0.415246442777429 -1.15554988401747]  x2=[1.26090477118469e-09 381852.398472139 381852.398472139;314.159265358979 314.159265358979 314.159265358979;-1.41941675517191 0.415007521738739 -1.15578880505616]  x3=[1.07663708898761e-11 1405.24743813465 1405.24743813466;314.159265358979 314.159265358979 314.159265358979;-2.70558821102223 0.316110507002444 -1.25468581979246]  x4=[8.62234243168895e-12 1405.96374414071 1405.9637441407;314.159265358979 314.159265358979 314.159265358979;0.245769282942371 0.405640215255436 -1.16515611153945]  x5=0.000565541566995742  V1=ones(3,3)  V2=ones(3,3)  I1=ones(3,3)  I2=ones(3,3)  nHarmo=1  Measurements=None
  _CN_92348290_765000_CN_167540668_765000 : powerlib/Elements/Distributed Parameters Line  Phases=3  Frequency=50  Resistance=[0.01273 0.3864]  Inductance="[0.9337e-3  4.1264e-3]"  Capacitance=[12.74e-9 7.751e-9]  Length=143.0094  x1=[8.73114913702011e-11 380000 380000;314.159265358979 314.159265358979 314.159265358979;-0.177670123217348 0.415246442777429 -1.15554988401747]  x2=[1.26090477118469e-09 381852.398472139 381852.398472139;314.159265358979 314.159265358979 314.159265358979;-1.41941675517191 0.415007521738739 -1.15578880505616]  x3=[1.07663708898761e-11 1405.24743813465 1405.24743813466;314.159265358979 314.159265358979 314.159265358979;-2.70558821102223 0.316110507002444 -1.25468581979246]  x4=[8.62234243168895e-12 1405.96374414071 1405.9637441407;314.159265358979 314.159265358979 314.159265358979;0.245769282942371 0.405640215255436 -1.16515611153945]  x5=0.000565541566995742  V1=ones(3,3)  V2=ones(3,3)  I1=ones(3,3)  I2=ones(3,3)  nHarmo=1  Measurements=None
  _CN_92348290_765000_CN_193977981_765000 : powerlib/Elements/Distributed Parameters Line  Phases=3  Frequency=50  Resistance=[0.01273 0.3864]  Inductance="[0.9337e-3  4.1264e-3]"  Capacitance=[12.74e-9 7.751e-9]  Length=294.817  x1=[8.73114913702011e-11 380000 380000;314.159265358979 314.159265358979 314.159265358979;-0.177670123217348 0.415246442777429 -1.15554988401747]  x2=[1.26090477118469e-09 381852.398472139 381852.398472139;314.159265358979 314.159265358979 314.159265358979;-1.41941675517191 0.415007521738739 -1.15578880505616]  x3=[1.07663708898761e-11 1405.24743813465 1405.24743813466;314.159265358979 314.159265358979 314.159265358979;-2.70558821102223 0.316110507002444 -1.25468581979246]  x4=[8.62234243168895e-12 1405.96374414071 1405.9637441407;314.159265358979 314.159265358979 314.159265358979;0.245769282942371 0.405640215255436 -1.16515611153945]  x5=0.000565541566995742  V1=ones(3,3)  V2=ones(3,3)  I1=ones(3,3)  I2=ones(3,3)  nHarmo=1  Measurements=None
  _CN_93158442_275000_CN_101150274_275000 : powerlib/Elements/Distributed Parameters Line  Phases=3  Frequency=50  Resistance=[0.01273 0.3864]  Inductance="[0.9337e-3  4.1264e-3]"  Capacitance=[12.74e-9 7.751e-9]  Length=91.3195  x1=[8.73114913702011e-11 380000 380000;314.159265358979 314.159265358979 314.159265358979;-0.177670123217348 0.415246442777429 -1.15554988401747]  x2=[1.26090477118469e-09 381852.398472139 381852.398472139;314.159265358979 314.159265358979 314.159265358979;-1.41941675517191 0.415007521738739 -1.15578880505616]  x3=[1.07663708898761e-11 1405.24743813465 1405.24743813466;314.159265358979 314.159265358979 314.159265358979;-2.70558821102223 0.316110507002444 -1.25468581979246]  x4=[8.62234243168895e-12 1405.96374414071 1405.9637441407;314.159265358979 314.159265358979 314.159265358979;0.245769282942371 0.405640215255436 -1.16515611153945]  x5=0.000565541566995742  V1=ones(3,3)  V2=ones(3,3)  I1=ones(3,3)  I2=ones(3,3)  nHarmo=1  Measurements=None
  _CN_98218556_400000_CN_185341297_400000 : powerlib/Elements/Distributed Parameters Line  Phases=3  Frequency=50  Resistance=[0.01273 0.3864]  Inductance="[0.9337e-3  4.1264e-3]"  Capacitance=[12.74e-9 7.751e-9]  Length=83.4269  x1=[8.73114913702011e-11 380000 380000;314.159265358979 314.159265358979 314.159265358979;-0.177670123217348 0.415246442777429 -1.15554988401747]  x2=[1.26090477118469e-09 381852.398472139 381852.398472139;314.159265358979 314.159265358979 314.159265358979;-1.41941675517191 0.415007521738739 -1.15578880505616]  x3=[1.07663708898761e-11 1405.24743813465 1405.24743813466;314.159265358979 314.159265358979 314.159265358979;-2.70558821102223 0.316110507002444 -1.25468581979246]  x4=[8.62234243168895e-12 1405.96374414071 1405.9637441407;314.159265358979 314.159265358979 314.159265358979;0.245769282942371 0.405640215255436 -1.16515611153945]  x5=0.000565541566995742  V1=ones(3,3)  V2=ones(3,3)  I1=ones(3,3)  I2=ones(3,3)  nHarmo=1  Measurements=None
  _CN_98231311_400000_CN_178968761_400000 : powerlib/Elements/Distributed Parameters Line  Phases=3  Frequency=50  Resistance=[0.01273 0.3864]  Inductance="[0.9337e-3  4.1264e-3]"  Capacitance=[12.74e-9 7.751e-9]  Length=61.9606  x1=[8.73114913702011e-11 380000 380000;314.159265358979 314.159265358979 314.159265358979;-0.177670123217348 0.415246442777429 -1.15554988401747]  x2=[1.26090477118469e-09 381852.398472139 381852.398472139;314.159265358979 314.159265358979 314.159265358979;-1.41941675517191 0.415007521738739 -1.15578880505616]  x3=[1.07663708898761e-11 1405.24743813465 1405.24743813466;314.159265358979 314.159265358979 314.159265358979;-2.70558821102223 0.316110507002444 -1.25468581979246]  x4=[8.62234243168895e-12 1405.96374414071 1405.9637441407;314.159265358979 314.159265358979 314.159265358979;0.245769282942371 0.405640215255436 -1.16515611153945]  x5=0.000565541566995742  V1=ones(3,3)  V2=ones(3,3)  I1=ones(3,3)  I2=ones(3,3)  nHarmo=1  Measurements=None
  _CN_98231311_400000_CN_386388564_400000 : powerlib/Elements/Distributed Parameters Line  Phases=3  Frequency=50  Resistance=[0.01273 0.3864]  Inductance="[0.9337e-3  4.1264e-3]"  Capacitance=[12.74e-9 7.751e-9]  Length=223.9155  x1=[8.73114913702011e-11 380000 380000;314.159265358979 314.159265358979 314.159265358979;-0.177670123217348 0.415246442777429 -1.15554988401747]  x2=[1.26090477118469e-09 381852.398472139 381852.398472139;314.159265358979 314.159265358979 314.159265358979;-1.41941675517191 0.415007521738739 -1.15578880505616]  x3=[1.07663708898761e-11 1405.24743813465 1405.24743813466;314.159265358979 314.159265358979 314.159265358979;-2.70558821102223 0.316110507002444 -1.25468581979246]  x4=[8.62234243168895e-12 1405.96374414071 1405.9637441407;314.159265358979 314.159265358979 314.159265358979;0.245769282942371 0.405640215255436 -1.16515611153945]  x5=0.000565541566995742  V1=ones(3,3)  V2=ones(3,3)  I1=ones(3,3)  I2=ones(3,3)  nHarmo=1  Measurements=None
  _CN_98231341_275000_CN_105811523_275000 : powerlib/Elements/Distributed Parameters Line  Phases=3  Frequency=50  Resistance=[0.01273 0.3864]  Inductance="[0.9337e-3  4.1264e-3]"  Capacitance=[12.74e-9 7.751e-9]  Length=21.1695  x1=[8.73114913702011e-11 380000 380000;314.159265358979 314.159265358979 314.159265358979;-0.177670123217348 0.415246442777429 -1.15554988401747]  x2=[1.26090477118469e-09 381852.398472139 381852.398472139;314.159265358979 314.159265358979 314.159265358979;-1.41941675517191 0.415007521738739 -1.15578880505616]  x3=[1.07663708898761e-11 1405.24743813465 1405.24743813466;314.159265358979 314.159265358979 314.159265358979;-2.70558821102223 0.316110507002444 -1.25468581979246]  x4=[8.62234243168895e-12 1405.96374414071 1405.9637441407;314.159265358979 314.159265358979 314.159265358979;0.245769282942371 0.405640215255436 -1.16515611153945]  x5=0.000565541566995742  V1=ones(3,3)  V2=ones(3,3)  I1=ones(3,3)  I2=ones(3,3)  nHarmo=1  Measurements=None
  _CN_98231341_275000_CN_136695854_275000 : powerlib/Elements/Distributed Parameters Line  Phases=3  Frequency=50  Resistance=[0.01273 0.3864]  Inductance="[0.9337e-3  4.1264e-3]"  Capacitance=[12.74e-9 7.751e-9]  Length=34.7453  x1=[8.73114913702011e-11 380000 380000;314.159265358979 314.159265358979 314.159265358979;-0.177670123217348 0.415246442777429 -1.15554988401747]  x2=[1.26090477118469e-09 381852.398472139 381852.398472139;314.159265358979 314.159265358979 314.159265358979;-1.41941675517191 0.415007521738739 -1.15578880505616]  x3=[1.07663708898761e-11 1405.24743813465 1405.24743813466;314.159265358979 314.159265358979 314.159265358979;-2.70558821102223 0.316110507002444 -1.25468581979246]  x4=[8.62234243168895e-12 1405.96374414071 1405.9637441407;314.159265358979 314.159265358979 314.159265358979;0.245769282942371 0.405640215255436 -1.16515611153945]  x5=0.000565541566995742  V1=ones(3,3)  V2=ones(3,3)  I1=ones(3,3)  I2=ones(3,3)  nHarmo=1  Measurements=None
  _CN_98231341_275000_CN_189739076_275000 : powerlib/Elements/Distributed Parameters Line  Phases=3  Frequency=50  Resistance=[0.01273 0.3864]  Inductance="[0.9337e-3  4.1264e-3]"  Capacitance=[12.74e-9 7.751e-9]  Length=13.5116  x1=[8.73114913702011e-11 380000 380000;314.159265358979 314.159265358979 314.159265358979;-0.177670123217348 0.415246442777429 -1.15554988401747]  x2=[1.26090477118469e-09 381852.398472139 381852.398472139;314.159265358979 314.159265358979 314.159265358979;-1.41941675517191 0.415007521738739 -1.15578880505616]  x3=[1.07663708898761e-11 1405.24743813465 1405.24743813466;314.159265358979 314.159265358979 314.159265358979;-2.70558821102223 0.316110507002444 -1.25468581979246]  x4=[8.62234243168895e-12 1405.96374414071 1405.9637441407;314.159265358979 314.159265358979 314.159265358979;0.245769282942371 0.405640215255436 -1.16515611153945]  x5=0.000565541566995742  V1=ones(3,3)  V2=ones(3,3)  I1=ones(3,3)  I2=ones(3,3)  nHarmo=1  Measurements=None
  _CN_98231341_275000_CN_214437948_275000 : powerlib/Elements/Distributed Parameters Line  Phases=3  Frequency=50  Resistance=[0.01273 0.3864]  Inductance="[0.9337e-3  4.1264e-3]"  Capacitance=[12.74e-9 7.751e-9]  Length=67.1874  x1=[8.73114913702011e-11 380000 380000;314.159265358979 314.159265358979 314.159265358979;-0.177670123217348 0.415246442777429 -1.15554988401747]  x2=[1.26090477118469e-09 381852.398472139 381852.398472139;314.159265358979 314.159265358979 314.159265358979;-1.41941675517191 0.415007521738739 -1.15578880505616]  x3=[1.07663708898761e-11 1405.24743813465 1405.24743813466;314.159265358979 314.159265358979 314.159265358979;-2.70558821102223 0.316110507002444 -1.25468581979246]  x4=[8.62234243168895e-12 1405.96374414071 1405.9637441407;314.159265358979 314.159265358979 314.159265358979;0.245769282942371 0.405640215255436 -1.16515611153945]  x5=0.000565541566995742  V1=ones(3,3)  V2=ones(3,3)  I1=ones(3,3)  I2=ones(3,3)  nHarmo=1  Measurements=None
  _CN_98231341_275000_CN_81817181_275000 : powerlib/Elements/Distributed Parameters Line  Phases=3  Frequency=50  Resistance=[0.01273 0.3864]  Inductance="[0.9337e-3  4.1264e-3]"  Capacitance=[12.74e-9 7.751e-9]  Length=61.7457  x1=[8.73114913702011e-11 380000 380000;314.159265358979 314.159265358979 314.159265358979;-0.177670123217348 0.415246442777429 -1.15554988401747]  x2=[1.26090477118469e-09 381852.398472139 381852.398472139;314.159265358979 314.159265358979 314.159265358979;-1.41941675517191 0.415007521738739 -1.15578880505616]  x3=[1.07663708898761e-11 1405.24743813465 1405.24743813466;314.159265358979 314.159265358979 314.159265358979;-2.70558821102223 0.316110507002444 -1.25468581979246]  x4=[8.62234243168895e-12 1405.96374414071 1405.9637441407;314.159265358979 314.159265358979 314.159265358979;0.245769282942371 0.405640215255436 -1.16515611153945]  x5=0.000565541566995742  V1=ones(3,3)  V2=ones(3,3)  I1=ones(3,3)  I2=ones(3,3)  nHarmo=1  Measurements=None
  bus1 : powerlib/Measurements/Load Flow Bus  LConnTagsString=a  Phases=single  Connectors=on one side  ID=bus1  Vbase=132000  Vref=1  Vangle=0  VLF=1  VLFb=1  VLFc=1  angleLF=0  angleLFb=0  angleLFc=0
      settings: AttributesFormatString=|
      | %<ID>
      | %<Vbase>V
      | %<VLF>pu
      | %<angleLF>deg.
      | %<Name>
  bus10 : powerlib/Measurements/Load Flow Bus  LConnTagsString=a  Phases=single  Connectors=on one side  ID=bus10  Vbase=132000  Vref=1  Vangle=0  VLF=1  VLFb=1  VLFc=1  angleLF=0  angleLFb=0  angleLFc=0
      settings: AttributesFormatString=|
      | %<ID>
      | %<Vbase>V
      | %<VLF>pu
      | %<angleLF>deg.
      | %<Name>
  bus100 : powerlib/Measurements/Load Flow Bus  LConnTagsString=a  Phases=single  Connectors=on one side  ID=bus100  Vbase=275000  Vref=1  Vangle=0  VLF=1  VLFb=1  VLFc=1  angleLF=0  angleLFb=0  angleLFc=0
      settings: AttributesFormatString=|
      | %<ID>
      | %<Vbase>V
      | %<VLF>pu
      | %<angleLF>deg.
      | %<Name>
  bus101 : powerlib/Measurements/Load Flow Bus  LConnTagsString=a  Phases=single  Connectors=on one side  ID=bus101  Vbase=275000  Vref=1  Vangle=0  VLF=1  VLFb=1  VLFc=1  angleLF=0  angleLFb=0  angleLFc=0
      settings: AttributesFormatString=|
      | %<ID>
      | %<Vbase>V
      | %<VLF>pu
      | %<angleLF>deg.
      | %<Name>
  bus102 : powerlib/Measurements/Load Flow Bus  LConnTagsString=a  Phases=single  Connectors=on one side  ID=bus102  Vbase=275000  Vref=1  Vangle=0  VLF=1  VLFb=1  VLFc=1  angleLF=0  angleLFb=0  angleLFc=0
      settings: AttributesFormatString=|
      | %<ID>
      | %<Vbase>V
      | %<VLF>pu
      | %<angleLF>deg.
      | %<Name>
  bus103 : powerlib/Measurements/Load Flow Bus  LConnTagsString=a  Phases=single  Connectors=on one side  ID=bus103  Vbase=275000  Vref=1  Vangle=0  VLF=1  VLFb=1  VLFc=1  angleLF=0  angleLFb=0  angleLFc=0
      settings: AttributesFormatString=|
      | %<ID>
      | %<Vbase>V
      | %<VLF>pu
      | %<angleLF>deg.
      | %<Name>
  bus104 : powerlib/Measurements/Load Flow Bus  LConnTagsString=a  Phases=single  Connectors=on one side  ID=bus104  Vbase=275000  Vref=1  Vangle=0  VLF=1  VLFb=1  VLFc=1  angleLF=0  angleLFb=0  angleLFc=0
      settings: AttributesFormatString=|
      | %<ID>
      | %<Vbase>V
      | %<VLF>pu
      | %<angleLF>deg.
      | %<Name>
  bus105 : powerlib/Measurements/Load Flow Bus  LConnTagsString=a  Phases=single  Connectors=on one side  ID=bus105  Vbase=275000  Vref=1  Vangle=0  VLF=1  VLFb=1  VLFc=1  angleLF=0  angleLFb=0  angleLFc=0
      settings: AttributesFormatString=|
      | %<ID>
      | %<Vbase>V
      | %<VLF>pu
      | %<angleLF>deg.
      | %<Name>
  bus106 : powerlib/Measurements/Load Flow Bus  LConnTagsString=a  Phases=single  Connectors=on one side  ID=bus106  Vbase=275000  Vref=1  Vangle=0  VLF=1  VLFb=1  VLFc=1  angleLF=0  angleLFb=0  angleLFc=0
      settings: AttributesFormatString=|
      | %<ID>
      | %<Vbase>V
      | %<VLF>pu
      | %<angleLF>deg.
      | %<Name>
  bus107 : powerlib/Measurements/Load Flow Bus  LConnTagsString=a  Phases=single  Connectors=on one side  ID=bus107  Vbase=275000  Vref=1  Vangle=0  VLF=1  VLFb=1  VLFc=1  angleLF=0  angleLFb=0  angleLFc=0
      settings: AttributesFormatString=|
      | %<ID>
      | %<Vbase>V
      | %<VLF>pu
      | %<angleLF>deg.
      | %<Name>
  bus108 : powerlib/Measurements/Load Flow Bus  LConnTagsString=a  Phases=single  Connectors=on one side  ID=bus108  Vbase=275000  Vref=1  Vangle=0  VLF=1  VLFb=1  VLFc=1  angleLF=0  angleLFb=0  angleLFc=0
      settings: AttributesFormatString=|
      | %<ID>
      | %<Vbase>V
      | %<VLF>pu
      | %<angleLF>deg.
      | %<Name>
  bus109 : powerlib/Measurements/Load Flow Bus  LConnTagsString=a  Phases=single  Connectors=on one side  ID=bus109  Vbase=275000  Vref=1  Vangle=0  VLF=1  VLFb=1  VLFc=1  angleLF=0  angleLFb=0  angleLFc=0
      settings: AttributesFormatString=|
      | %<ID>
      | %<Vbase>V
      | %<VLF>pu
      | %<angleLF>deg.
      | %<Name>
  bus11 : powerlib/Measurements/Load Flow Bus  LConnTagsString=a  Phases=single  Connectors=on one side  ID=bus11  Vbase=132000  Vref=1  Vangle=0  VLF=1  VLFb=1  VLFc=1  angleLF=0  angleLFb=0  angleLFc=0
      settings: AttributesFormatString=|
      | %<ID>
      | %<Vbase>V
      | %<VLF>pu
      | %<angleLF>deg.
      | %<Name>
  bus110 : powerlib/Measurements/Load Flow Bus  LConnTagsString=a  Phases=single  Connectors=on one side  ID=bus110  Vbase=275000  Vref=1  Vangle=0  VLF=1  VLFb=1  VLFc=1  angleLF=0  angleLFb=0  angleLFc=0
      settings: AttributesFormatString=|
      | %<ID>
      | %<Vbase>V
      | %<VLF>pu
      | %<angleLF>deg.
      | %<Name>
  bus111 : powerlib/Measurements/Load Flow Bus  LConnTagsString=a  Phases=single  Connectors=on one side  ID=bus111  Vbase=275000  Vref=1  Vangle=0  VLF=1  VLFb=1  VLFc=1  angleLF=0  angleLFb=0  angleLFc=0
      settings: AttributesFormatString=|
      | %<ID>
      | %<Vbase>V
      | %<VLF>pu
      | %<angleLF>deg.
      | %<Name>
  bus112 : powerlib/Measurements/Load Flow Bus  LConnTagsString=a  Phases=single  Connectors=on one side  ID=bus112  Vbase=275000  Vref=1  Vangle=0  VLF=1  VLFb=1  VLFc=1  angleLF=0  angleLFb=0  angleLFc=0
      settings: AttributesFormatString=|
      | %<ID>
      | %<Vbase>V
      | %<VLF>pu
      | %<angleLF>deg.
      | %<Name>
  bus113 : powerlib/Measurements/Load Flow Bus  LConnTagsString=a  Phases=single  Connectors=on one side  ID=bus113  Vbase=275000  Vref=1  Vangle=0  VLF=1  VLFb=1  VLFc=1  angleLF=0  angleLFb=0  angleLFc=0
      settings: AttributesFormatString=|
      | %<ID>
      | %<Vbase>V
      | %<VLF>pu
      | %<angleLF>deg.
      | %<Name>
  bus114 : powerlib/Measurements/Load Flow Bus  LConnTagsString=a  Phases=single  Connectors=on one side  ID=bus114  Vbase=275000  Vref=1  Vangle=0  VLF=1  VLFb=1  VLFc=1  angleLF=0  angleLFb=0  angleLFc=0
      settings: AttributesFormatString=|
      | %<ID>
      | %<Vbase>V
      | %<VLF>pu
      | %<angleLF>deg.
      | %<Name>
  bus115 : powerlib/Measurements/Load Flow Bus  LConnTagsString=a  Phases=single  Connectors=on one side  ID=bus115  Vbase=275000  Vref=1  Vangle=0  VLF=1  VLFb=1  VLFc=1  angleLF=0  angleLFb=0  angleLFc=0
      settings: AttributesFormatString=|
      | %<ID>
      | %<Vbase>V
      | %<VLF>pu
      | %<angleLF>deg.
      | %<Name>
  bus116 : powerlib/Measurements/Load Flow Bus  LConnTagsString=a  Phases=single  Connectors=on one side  ID=bus116  Vbase=275000  Vref=1  Vangle=0  VLF=1  VLFb=1  VLFc=1  angleLF=0  angleLFb=0  angleLFc=0
      settings: AttributesFormatString=|
      | %<ID>
      | %<Vbase>V
      | %<VLF>pu
      | %<angleLF>deg.
      | %<Name>
  bus117 : powerlib/Measurements/Load Flow Bus  LConnTagsString=a  Phases=single  Connectors=on one side  ID=bus117  Vbase=275000  Vref=1  Vangle=0  VLF=1  VLFb=1  VLFc=1  angleLF=0  angleLFb=0  angleLFc=0
      settings: AttributesFormatString=|
      | %<ID>
      | %<Vbase>V
      | %<VLF>pu
      | %<angleLF>deg.
      | %<Name>
  bus118 : powerlib/Measurements/Load Flow Bus  LConnTagsString=a  Phases=single  Connectors=on one side  ID=bus118  Vbase=275000  Vref=1  Vangle=0  VLF=1  VLFb=1  VLFc=1  angleLF=0  angleLFb=0  angleLFc=0
      settings: AttributesFormatString=|
      | %<ID>
      | %<Vbase>V
      | %<VLF>pu
      | %<angleLF>deg.
      | %<Name>
  bus119 : powerlib/Measurements/Load Flow Bus  LConnTagsString=a  Phases=single  Connectors=on one side  ID=bus119  Vbase=275000  Vref=1  Vangle=0  VLF=1  VLFb=1  VLFc=1  angleLF=0  angleLFb=0  angleLFc=0
      settings: AttributesFormatString=|
      | %<ID>
      | %<Vbase>V
      | %<VLF>pu
      | %<angleLF>deg.
      | %<Name>
  bus12 : powerlib/Measurements/Load Flow Bus  LConnTagsString=a  Phases=single  Connectors=on one side  ID=bus12  Vbase=132000  Vref=1  Vangle=0  VLF=1  VLFb=1  VLFc=1  angleLF=0  angleLFb=0  angleLFc=0
      settings: AttributesFormatString=|
      | %<ID>
      | %<Vbase>V
      | %<VLF>pu
      | %<angleLF>deg.
      | %<Name>
  bus120 : powerlib/Measurements/Load Flow Bus  LConnTagsString=a  Phases=single  Connectors=on one side  ID=bus120  Vbase=275000  Vref=1  Vangle=0  VLF=1  VLFb=1  VLFc=1  angleLF=0  angleLFb=0  angleLFc=0
      settings: AttributesFormatString=|
      | %<ID>
      | %<Vbase>V
      | %<VLF>pu
      | %<angleLF>deg.
      | %<Name>
  bus121 : powerlib/Measurements/Load Flow Bus  LConnTagsString=a  Phases=single  Connectors=on one side  ID=bus121  Vbase=275000  Vref=1  Vangle=0  VLF=1  VLFb=1  VLFc=1  angleLF=0  angleLFb=0  angleLFc=0
      settings: AttributesFormatString=|
      | %<ID>
      | %<Vbase>V
      | %<VLF>pu
      | %<angleLF>deg.
      | %<Name>
  bus122 : powerlib/Measurements/Load Flow Bus  LConnTagsString=a  Phases=single  Connectors=on one side  ID=bus122  Vbase=275000  Vref=1  Vangle=0  VLF=1  VLFb=1  VLFc=1  angleLF=0  angleLFb=0  angleLFc=0
      settings: AttributesFormatString=|
      | %<ID>
      | %<Vbase>V
      | %<VLF>pu
      | %<angleLF>deg.
      | %<Name>
  bus123 : powerlib/Measurements/Load Flow Bus  LConnTagsString=a  Phases=single  Connectors=on one side  ID=bus123  Vbase=275000  Vref=1  Vangle=0  VLF=1  VLFb=1  VLFc=1  angleLF=0  angleLFb=0  angleLFc=0
      settings: AttributesFormatString=|
      | %<ID>
      | %<Vbase>V
      | %<VLF>pu
      | %<angleLF>deg.
      | %<Name>
  bus124 : powerlib/Measurements/Load Flow Bus  LConnTagsString=a  Phases=single  Connectors=on one side  ID=bus124  Vbase=275000  Vref=1  Vangle=0  VLF=1  VLFb=1  VLFc=1  angleLF=0  angleLFb=0  angleLFc=0
      settings: AttributesFormatString=|
      | %<ID>
      | %<Vbase>V
      | %<VLF>pu
      | %<angleLF>deg.
      | %<Name>
  bus125 : powerlib/Measurements/Load Flow Bus  LConnTagsString=a  Phases=single  Connectors=on one side  ID=bus125  Vbase=275000  Vref=1  Vangle=0  VLF=1  VLFb=1  VLFc=1  angleLF=0  angleLFb=0  angleLFc=0
      settings: AttributesFormatString=|
      | %<ID>
      | %<Vbase>V
      | %<VLF>pu
      | %<angleLF>deg.
      | %<Name>
  bus126 : powerlib/Measurements/Load Flow Bus  LConnTagsString=a  Phases=single  Connectors=on one side  ID=bus126  Vbase=275000  Vref=1  Vangle=0  VLF=1  VLFb=1  VLFc=1  angleLF=0  angleLFb=0  angleLFc=0
      settings: AttributesFormatString=|
      | %<ID>
      | %<Vbase>V
      | %<VLF>pu
      | %<angleLF>deg.
      | %<Name>
  bus127 : powerlib/Measurements/Load Flow Bus  LConnTagsString=a  Phases=single  Connectors=on one side  ID=bus127  Vbase=275000  Vref=1  Vangle=0  VLF=1  VLFb=1  VLFc=1  angleLF=0  angleLFb=0  angleLFc=0
      settings: AttributesFormatString=|
      | %<ID>
      | %<Vbase>V
      | %<VLF>pu
      | %<angleLF>deg.
      | %<Name>
  bus128 : powerlib/Measurements/Load Flow Bus  LConnTagsString=a  Phases=single  Connectors=on one side  ID=bus128  Vbase=275000  Vref=1  Vangle=0  VLF=1  VLFb=1  VLFc=1  angleLF=0  angleLFb=0  angleLFc=0
      settings: AttributesFormatString=|
      | %<ID>
      | %<Vbase>V
      | %<VLF>pu
      | %<angleLF>deg.
      | %<Name>
  bus129 : powerlib/Measurements/Load Flow Bus  LConnTagsString=a  Phases=single  Connectors=on one side  ID=bus129  Vbase=275000  Vref=1  Vangle=0  VLF=1  VLFb=1  VLFc=1  angleLF=0  angleLFb=0  angleLFc=0
      settings: AttributesFormatString=|
      | %<ID>
      | %<Vbase>V
      | %<VLF>pu
      | %<angleLF>deg.
      | %<Name>
  bus13 : powerlib/Measurements/Load Flow Bus  LConnTagsString=a  Phases=single  Connectors=on one side  ID=bus13  Vbase=132000  Vref=1  Vangle=0  VLF=1  VLFb=1  VLFc=1  angleLF=0  angleLFb=0  angleLFc=0
      settings: AttributesFormatString=|
      | %<ID>
      | %<Vbase>V
      | %<VLF>pu
      | %<angleLF>deg.
      | %<Name>
  bus130 : powerlib/Measurements/Load Flow Bus  LConnTagsString=a  Phases=single  Connectors=on one side  ID=bus130  Vbase=275000  Vref=1  Vangle=0  VLF=1  VLFb=1  VLFc=1  angleLF=0  angleLFb=0  angleLFc=0
      settings: AttributesFormatString=|
      | %<ID>
      | %<Vbase>V
      | %<VLF>pu
      | %<angleLF>deg.
      | %<Name>
  bus131 : powerlib/Measurements/Load Flow Bus  LConnTagsString=a  Phases=single  Connectors=on one side  ID=bus131  Vbase=275000  Vref=1  Vangle=0  VLF=1  VLFb=1  VLFc=1  angleLF=0  angleLFb=0  angleLFc=0
      settings: AttributesFormatString=|
      | %<ID>
      | %<Vbase>V
      | %<VLF>pu
      | %<angleLF>deg.
      | %<Name>
  bus132 : powerlib/Measurements/Load Flow Bus  LConnTagsString=a  Phases=single  Connectors=on one side  ID=bus132  Vbase=275000  Vref=1  Vangle=0  VLF=1  VLFb=1  VLFc=1  angleLF=0  angleLFb=0  angleLFc=0
      settings: AttributesFormatString=|
      | %<ID>
      | %<Vbase>V
      | %<VLF>pu
      | %<angleLF>deg.
      | %<Name>
  bus133 : powerlib/Measurements/Load Flow Bus  LConnTagsString=a  Phases=single  Connectors=on one side  ID=bus133  Vbase=275000  Vref=1  Vangle=0  VLF=1  VLFb=1  VLFc=1  angleLF=0  angleLFb=0  angleLFc=0
      settings: AttributesFormatString=|
      | %<ID>
      | %<Vbase>V
      | %<VLF>pu
      | %<angleLF>deg.
      | %<Name>
  bus134 : powerlib/Measurements/Load Flow Bus  LConnTagsString=a  Phases=single  Connectors=on one side  ID=bus134  Vbase=275000  Vref=1  Vangle=0  VLF=1  VLFb=1  VLFc=1  angleLF=0  angleLFb=0  angleLFc=0
      settings: AttributesFormatString=|
      | %<ID>
      | %<Vbase>V
      | %<VLF>pu
      | %<angleLF>deg.
      | %<Name>
  bus135 : powerlib/Measurements/Load Flow Bus  LConnTagsString=a  Phases=single  Connectors=on one side  ID=bus135  Vbase=275000  Vref=1  Vangle=0  VLF=1  VLFb=1  VLFc=1  angleLF=0  angleLFb=0  angleLFc=0
      settings: AttributesFormatString=|
      | %<ID>
      | %<Vbase>V
      | %<VLF>pu
      | %<angleLF>deg.
      | %<Name>
  bus136 : powerlib/Measurements/Load Flow Bus  LConnTagsString=a  Phases=single  Connectors=on one side  ID=bus136  Vbase=275000  Vref=1  Vangle=0  VLF=1  VLFb=1  VLFc=1  angleLF=0  angleLFb=0  angleLFc=0
      settings: AttributesFormatString=|
      | %<ID>
      | %<Vbase>V
      | %<VLF>pu
      | %<angleLF>deg.
      | %<Name>
  bus137 : powerlib/Measurements/Load Flow Bus  LConnTagsString=a  Phases=single  Connectors=on one side  ID=bus137  Vbase=275000  Vref=1  Vangle=0  VLF=1  VLFb=1  VLFc=1  angleLF=0  angleLFb=0  angleLFc=0
      settings: AttributesFormatString=|
      | %<ID>
      | %<Vbase>V
      | %<VLF>pu
      | %<angleLF>deg.
      | %<Name>
  bus138 : powerlib/Measurements/Load Flow Bus  LConnTagsString=a  Phases=single  Connectors=on one side  ID=bus138  Vbase=275000  Vref=1  Vangle=0  VLF=1  VLFb=1  VLFc=1  angleLF=0  angleLFb=0  angleLFc=0
      settings: AttributesFormatString=|
      | %<ID>
      | %<Vbase>V
      | %<VLF>pu
      | %<angleLF>deg.
      | %<Name>
  bus139 : powerlib/Measurements/Load Flow Bus  LConnTagsString=a  Phases=single  Connectors=on one side  ID=bus139  Vbase=275000  Vref=1  Vangle=0  VLF=1  VLFb=1  VLFc=1  angleLF=0  angleLFb=0  angleLFc=0
      settings: AttributesFormatString=|
      | %<ID>
      | %<Vbase>V
      | %<VLF>pu
      | %<angleLF>deg.
      | %<Name>
  bus14 : powerlib/Measurements/Load Flow Bus  LConnTagsString=a  Phases=single  Connectors=on one side  ID=bus14  Vbase=132000  Vref=1  Vangle=0  VLF=1  VLFb=1  VLFc=1  angleLF=0  angleLFb=0  angleLFc=0
      settings: AttributesFormatString=|
      | %<ID>
      | %<Vbase>V
      | %<VLF>pu
      | %<angleLF>deg.
      | %<Name>
  bus140 : powerlib/Measurements/Load Flow Bus  LConnTagsString=a  Phases=single  Connectors=on one side  ID=bus140  Vbase=275000  Vref=1  Vangle=0  VLF=1  VLFb=1  VLFc=1  angleLF=0  angleLFb=0  angleLFc=0
      settings: AttributesFormatString=|
      | %<ID>
      | %<Vbase>V
      | %<VLF>pu
      | %<angleLF>deg.
      | %<Name>
  bus141 : powerlib/Measurements/Load Flow Bus  LConnTagsString=a  Phases=single  Connectors=on one side  ID=bus141  Vbase=275000  Vref=1  Vangle=0  VLF=1  VLFb=1  VLFc=1  angleLF=0  angleLFb=0  angleLFc=0
      settings: AttributesFormatString=|
      | %<ID>
      | %<Vbase>V
      | %<VLF>pu
      | %<angleLF>deg.
      | %<Name>
  bus142 : powerlib/Measurements/Load Flow Bus  LConnTagsString=a  Phases=single  Connectors=on one side  ID=bus142  Vbase=275000  Vref=1  Vangle=0  VLF=1  VLFb=1  VLFc=1  angleLF=0  angleLFb=0  angleLFc=0
      settings: AttributesFormatString=|
      | %<ID>
      | %<Vbase>V
      | %<VLF>pu
      | %<angleLF>deg.
      | %<Name>
  bus143 : powerlib/Measurements/Load Flow Bus  LConnTagsString=a  Phases=single  Connectors=on one side  ID=bus143  Vbase=275000  Vref=1  Vangle=0  VLF=1  VLFb=1  VLFc=1  angleLF=0  angleLFb=0  angleLFc=0
      settings: AttributesFormatString=|
      | %<ID>
      | %<Vbase>V
      | %<VLF>pu
      | %<angleLF>deg.
      | %<Name>
  bus144 : powerlib/Measurements/Load Flow Bus  LConnTagsString=a  Phases=single  Connectors=on one side  ID=bus144  Vbase=275000  Vref=1  Vangle=0  VLF=1  VLFb=1  VLFc=1  angleLF=0  angleLFb=0  angleLFc=0
      settings: AttributesFormatString=|
      | %<ID>
      | %<Vbase>V
      | %<VLF>pu
      | %<angleLF>deg.
      | %<Name>
  bus145 : powerlib/Measurements/Load Flow Bus  LConnTagsString=a  Phases=single  Connectors=on one side  ID=bus145  Vbase=275000  Vref=1  Vangle=0  VLF=1  VLFb=1  VLFc=1  angleLF=0  angleLFb=0  angleLFc=0
      settings: AttributesFormatString=|
      | %<ID>
      | %<Vbase>V
      | %<VLF>pu
      | %<angleLF>deg.
      | %<Name>
  bus146 : powerlib/Measurements/Load Flow Bus  LConnTagsString=a  Phases=single  Connectors=on one side  ID=bus146  Vbase=275000  Vref=1  Vangle=0  VLF=1  VLFb=1  VLFc=1  angleLF=0  angleLFb=0  angleLFc=0
      settings: AttributesFormatString=|
      | %<ID>
      | %<Vbase>V
      | %<VLF>pu
      | %<angleLF>deg.
      | %<Name>
  bus147 : powerlib/Measurements/Load Flow Bus  LConnTagsString=a  Phases=single  Connectors=on one side  ID=bus147  Vbase=275000  Vref=1  Vangle=0  VLF=1  VLFb=1  VLFc=1  angleLF=0  angleLFb=0  angleLFc=0
      settings: AttributesFormatString=|
      | %<ID>
      | %<Vbase>V
      | %<VLF>pu
      | %<angleLF>deg.
      | %<Name>
  bus148 : powerlib/Measurements/Load Flow Bus  LConnTagsString=a  Phases=single  Connectors=on one side  ID=bus148  Vbase=275000  Vref=1  Vangle=0  VLF=1  VLFb=1  VLFc=1  angleLF=0  angleLFb=0  angleLFc=0
      settings: AttributesFormatString=|
      | %<ID>
      | %<Vbase>V
      | %<VLF>pu
      | %<angleLF>deg.
      | %<Name>
  bus149 : powerlib/Measurements/Load Flow Bus  LConnTagsString=a  Phases=single  Connectors=on one side  ID=bus149  Vbase=275000  Vref=1  Vangle=0  VLF=1  VLFb=1  VLFc=1  angleLF=0  angleLFb=0  angleLFc=0
      settings: AttributesFormatString=|
      | %<ID>
      | %<Vbase>V
      | %<VLF>pu
      | %<angleLF>deg.
      | %<Name>
  bus15 : powerlib/Measurements/Load Flow Bus  LConnTagsString=a  Phases=single  Connectors=on one side  ID=bus15  Vbase=132000  Vref=1  Vangle=0  VLF=1  VLFb=1  VLFc=1  angleLF=0  angleLFb=0  angleLFc=0
      settings: AttributesFormatString=|
      | %<ID>
      | %<Vbase>V
      | %<VLF>pu
      | %<angleLF>deg.
      | %<Name>
  bus150 : powerlib/Measurements/Load Flow Bus  LConnTagsString=a  Phases=single  Connectors=on one side  ID=bus150  Vbase=275000  Vref=1  Vangle=0  VLF=1  VLFb=1  VLFc=1  angleLF=0  angleLFb=0  angleLFc=0
      settings: AttributesFormatString=|
      | %<ID>
      | %<Vbase>V
      | %<VLF>pu
      | %<angleLF>deg.
      | %<Name>
  bus151 : powerlib/Measurements/Load Flow Bus  LConnTagsString=a  Phases=single  Connectors=on one side  ID=bus151  Vbase=275000  Vref=1  Vangle=0  VLF=1  VLFb=1  VLFc=1  angleLF=0  angleLFb=0  angleLFc=0
      settings: AttributesFormatString=|
      | %<ID>
      | %<Vbase>V
      | %<VLF>pu
      | %<angleLF>deg.
      | %<Name>
  bus152 : powerlib/Measurements/Load Flow Bus  LConnTagsString=a  Phases=single  Connectors=on one side  ID=bus152  Vbase=275000  Vref=1  Vangle=0  VLF=1  VLFb=1  VLFc=1  angleLF=0  angleLFb=0  angleLFc=0
      settings: AttributesFormatString=|
      | %<ID>
      | %<Vbase>V
      | %<VLF>pu
      | %<angleLF>deg.
      | %<Name>
  bus153 : powerlib/Measurements/Load Flow Bus  LConnTagsString=a  Phases=single  Connectors=on one side  ID=bus153  Vbase=275000  Vref=1  Vangle=0  VLF=1  VLFb=1  VLFc=1  angleLF=0  angleLFb=0  angleLFc=0
      settings: AttributesFormatString=|
      | %<ID>
      | %<Vbase>V
      | %<VLF>pu
      | %<angleLF>deg.
      | %<Name>
  bus154 : powerlib/Measurements/Load Flow Bus  LConnTagsString=a  Phases=single  Connectors=on one side  ID=bus154  Vbase=275000  Vref=1  Vangle=0  VLF=1  VLFb=1  VLFc=1  angleLF=0  angleLFb=0  angleLFc=0
      settings: AttributesFormatString=|
      | %<ID>
      | %<Vbase>V
      | %<VLF>pu
      | %<angleLF>deg.
      | %<Name>
  bus155 : powerlib/Measurements/Load Flow Bus  LConnTagsString=a  Phases=single  Connectors=on one side  ID=bus155  Vbase=275000  Vref=1  Vangle=0  VLF=1  VLFb=1  VLFc=1  angleLF=0  angleLFb=0  angleLFc=0
      settings: AttributesFormatString=|
      | %<ID>
      | %<Vbase>V
      | %<VLF>pu
      | %<angleLF>deg.
      | %<Name>
  bus156 : powerlib/Measurements/Load Flow Bus  LConnTagsString=a  Phases=single  Connectors=on one side  ID=bus156  Vbase=275000  Vref=1  Vangle=0  VLF=1  VLFb=1  VLFc=1  angleLF=0  angleLFb=0  angleLFc=0
      settings: AttributesFormatString=|
      | %<ID>
      | %<Vbase>V
      | %<VLF>pu
      | %<angleLF>deg.
      | %<Name>
  bus157 : powerlib/Measurements/Load Flow Bus  LConnTagsString=a  Phases=single  Connectors=on one side  ID=bus157  Vbase=275000  Vref=1  Vangle=0  VLF=1  VLFb=1  VLFc=1  angleLF=0  angleLFb=0  angleLFc=0
      settings: AttributesFormatString=|
      | %<ID>
      | %<Vbase>V
      | %<VLF>pu
      | %<angleLF>deg.
      | %<Name>
  bus158 : powerlib/Measurements/Load Flow Bus  LConnTagsString=a  Phases=single  Connectors=on one side  ID=bus158  Vbase=275000  Vref=1  Vangle=0  VLF=1  VLFb=1  VLFc=1  angleLF=0  angleLFb=0  angleLFc=0
      settings: AttributesFormatString=|
      | %<ID>
      | %<Vbase>V
      | %<VLF>pu
      | %<angleLF>deg.
      | %<Name>
  bus159 : powerlib/Measurements/Load Flow Bus  LConnTagsString=a  Phases=single  Connectors=on one side  ID=bus159  Vbase=275000  Vref=1  Vangle=0  VLF=1  VLFb=1  VLFc=1  angleLF=0  angleLFb=0  angleLFc=0
      settings: AttributesFormatString=|
      | %<ID>
      | %<Vbase>V
      | %<VLF>pu
      | %<angleLF>deg.
      | %<Name>
  bus16 : powerlib/Measurements/Load Flow Bus  LConnTagsString=a  Phases=single  Connectors=on one side  ID=bus16  Vbase=132000  Vref=1  Vangle=0  VLF=1  VLFb=1  VLFc=1  angleLF=0  angleLFb=0  angleLFc=0
      settings: AttributesFormatString=|
      | %<ID>
      | %<Vbase>V
      | %<VLF>pu
      | %<angleLF>deg.
      | %<Name>
  bus160 : powerlib/Measurements/Load Flow Bus  LConnTagsString=a  Phases=single  Connectors=on one side  ID=bus160  Vbase=275000  Vref=1  Vangle=0  VLF=1  VLFb=1  VLFc=1  angleLF=0  angleLFb=0  angleLFc=0
      settings: AttributesFormatString=|
      | %<ID>
      | %<Vbase>V
      | %<VLF>pu
      | %<angleLF>deg.
      | %<Name>
  bus161 : powerlib/Measurements/Load Flow Bus  LConnTagsString=a  Phases=single  Connectors=on one side  ID=bus161  Vbase=275000  Vref=1  Vangle=0  VLF=1  VLFb=1  VLFc=1  angleLF=0  angleLFb=0  angleLFc=0
      settings: AttributesFormatString=|
      | %<ID>
      | %<Vbase>V
      | %<VLF>pu
      | %<angleLF>deg.
      | %<Name>
  bus162 : powerlib/Measurements/Load Flow Bus  LConnTagsString=a  Phases=single  Connectors=on one side  ID=bus162  Vbase=275000  Vref=1  Vangle=0  VLF=1  VLFb=1  VLFc=1  angleLF=0  angleLFb=0  angleLFc=0
      settings: AttributesFormatString=|
      | %<ID>
      | %<Vbase>V
      | %<VLF>pu
      | %<angleLF>deg.
      | %<Name>
  bus163 : powerlib/Measurements/Load Flow Bus  LConnTagsString=a  Phases=single  Connectors=on one side  ID=bus163  Vbase=275000  Vref=1  Vangle=0  VLF=1  VLFb=1  VLFc=1  angleLF=0  angleLFb=0  angleLFc=0
      settings: AttributesFormatString=|
      | %<ID>
      | %<Vbase>V
      | %<VLF>pu
      | %<angleLF>deg.
      | %<Name>
  bus164 : powerlib/Measurements/Load Flow Bus  LConnTagsString=a  Phases=single  Connectors=on one side  ID=bus164  Vbase=275000  Vref=1  Vangle=0  VLF=1  VLFb=1  VLFc=1  angleLF=0  angleLFb=0  angleLFc=0
      settings: AttributesFormatString=|
      | %<ID>
      | %<Vbase>V
      | %<VLF>pu
      | %<angleLF>deg.
      | %<Name>
  bus165 : powerlib/Measurements/Load Flow Bus  LConnTagsString=a  Phases=single  Connectors=on one side  ID=bus165  Vbase=275000  Vref=1  Vangle=0  VLF=1  VLFb=1  VLFc=1  angleLF=0  angleLFb=0  angleLFc=0
      settings: AttributesFormatString=|
      | %<ID>
      | %<Vbase>V
      | %<VLF>pu
      | %<angleLF>deg.
      | %<Name>
  bus166 : powerlib/Measurements/Load Flow Bus  LConnTagsString=a  Phases=single  Connectors=on one side  ID=bus166  Vbase=275000  Vref=1  Vangle=0  VLF=1  VLFb=1  VLFc=1  angleLF=0  angleLFb=0  angleLFc=0
      settings: AttributesFormatString=|
      | %<ID>
      | %<Vbase>V
      | %<VLF>pu
      | %<angleLF>deg.
      | %<Name>
  bus167 : powerlib/Measurements/Load Flow Bus  LConnTagsString=a  Phases=single  Connectors=on one side  ID=bus167  Vbase=275000  Vref=1  Vangle=0  VLF=1  VLFb=1  VLFc=1  angleLF=0  angleLFb=0  angleLFc=0
      settings: AttributesFormatString=|
      | %<ID>
      | %<Vbase>V
      | %<VLF>pu
      | %<angleLF>deg.
      | %<Name>
  bus168 : powerlib/Measurements/Load Flow Bus  LConnTagsString=a  Phases=single  Connectors=on one side  ID=bus168  Vbase=275000  Vref=1  Vangle=0  VLF=1  VLFb=1  VLFc=1  angleLF=0  angleLFb=0  angleLFc=0
      settings: AttributesFormatString=|
      | %<ID>
      | %<Vbase>V
      | %<VLF>pu
      | %<angleLF>deg.
      | %<Name>
  bus169 : powerlib/Measurements/Load Flow Bus  LConnTagsString=a  Phases=single  Connectors=on one side  ID=bus169  Vbase=275000  Vref=1  Vangle=0  VLF=1  VLFb=1  VLFc=1  angleLF=0  angleLFb=0  angleLFc=0
      settings: AttributesFormatString=|
      | %<ID>
      | %<Vbase>V
      | %<VLF>pu
      | %<angleLF>deg.
      | %<Name>
  bus17 : powerlib/Measurements/Load Flow Bus  LConnTagsString=a  Phases=single  Connectors=on one side  ID=bus17  Vbase=132000  Vref=1  Vangle=0  VLF=1  VLFb=1  VLFc=1  angleLF=0  angleLFb=0  angleLFc=0
      settings: AttributesFormatString=|
      | %<ID>
      | %<Vbase>V
      | %<VLF>pu
      | %<angleLF>deg.
      | %<Name>
  bus170 : powerlib/Measurements/Load Flow Bus  LConnTagsString=a  Phases=single  Connectors=on one side  ID=bus170  Vbase=275000  Vref=1  Vangle=0  VLF=1  VLFb=1  VLFc=1  angleLF=0  angleLFb=0  angleLFc=0
      settings: AttributesFormatString=|
      | %<ID>
      | %<Vbase>V
      | %<VLF>pu
      | %<angleLF>deg.
      | %<Name>
  bus171 : powerlib/Measurements/Load Flow Bus  LConnTagsString=a  Phases=single  Connectors=on one side  ID=bus171  Vbase=275000  Vref=1  Vangle=0  VLF=1  VLFb=1  VLFc=1  angleLF=0  angleLFb=0  angleLFc=0
      settings: AttributesFormatString=|
      | %<ID>
      | %<Vbase>V
      | %<VLF>pu
      | %<angleLF>deg.
      | %<Name>
  bus172 : powerlib/Measurements/Load Flow Bus  LConnTagsString=a  Phases=single  Connectors=on one side  ID=bus172  Vbase=275000  Vref=1  Vangle=0  VLF=1  VLFb=1  VLFc=1  angleLF=0  angleLFb=0  angleLFc=0
      settings: AttributesFormatString=|
      | %<ID>
      | %<Vbase>V
      | %<VLF>pu
      | %<angleLF>deg.
      | %<Name>
  bus173 : powerlib/Measurements/Load Flow Bus  LConnTagsString=a  Phases=single  Connectors=on one side  ID=bus173  Vbase=275000  Vref=1  Vangle=0  VLF=1  VLFb=1  VLFc=1  angleLF=0  angleLFb=0  angleLFc=0
      settings: AttributesFormatString=|
      | %<ID>
      | %<Vbase>V
      | %<VLF>pu
      | %<angleLF>deg.
      | %<Name>
  bus174 : powerlib/Measurements/Load Flow Bus  LConnTagsString=a  Phases=single  Connectors=on one side  ID=bus174  Vbase=275000  Vref=1  Vangle=0  VLF=1  VLFb=1  VLFc=1  angleLF=0  angleLFb=0  angleLFc=0
      settings: AttributesFormatString=|
      | %<ID>
      | %<Vbase>V
      | %<VLF>pu
      | %<angleLF>deg.
      | %<Name>
  bus175 : powerlib/Measurements/Load Flow Bus  LConnTagsString=a  Phases=single  Connectors=on one side  ID=bus175  Vbase=275000  Vref=1  Vangle=0  VLF=1  VLFb=1  VLFc=1  angleLF=0  angleLFb=0  angleLFc=0
      settings: AttributesFormatString=|
      | %<ID>
      | %<Vbase>V
      | %<VLF>pu
      | %<angleLF>deg.
      | %<Name>
  bus176 : powerlib/Measurements/Load Flow Bus  LConnTagsString=a  Phases=single  Connectors=on one side  ID=bus176  Vbase=400000  Vref=1  Vangle=0  VLF=1  VLFb=1  VLFc=1  angleLF=0  angleLFb=0  angleLFc=0
      settings: AttributesFormatString=|
      | %<ID>
      | %<Vbase>V
      | %<VLF>pu
      | %<angleLF>deg.
      | %<Name>
  bus177 : powerlib/Measurements/Load Flow Bus  LConnTagsString=a  Phases=single  Connectors=on one side  ID=bus177  Vbase=400000  Vref=1  Vangle=0  VLF=1  VLFb=1  VLFc=1  angleLF=0  angleLFb=0  angleLFc=0
      settings: AttributesFormatString=|
      | %<ID>
      | %<Vbase>V
      | %<VLF>pu
      | %<angleLF>deg.
      | %<Name>
  bus178 : powerlib/Measurements/Load Flow Bus  LConnTagsString=a  Phases=single  Connectors=on one side  ID=bus178  Vbase=400000  Vref=1  Vangle=0  VLF=1  VLFb=1  VLFc=1  angleLF=0  angleLFb=0  angleLFc=0
      settings: AttributesFormatString=|
      | %<ID>
      | %<Vbase>V
      | %<VLF>pu
      | %<angleLF>deg.
      | %<Name>
  bus179 : powerlib/Measurements/Load Flow Bus  LConnTagsString=a  Phases=single  Connectors=on one side  ID=bus179  Vbase=400000  Vref=1  Vangle=0  VLF=1  VLFb=1  VLFc=1  angleLF=0  angleLFb=0  angleLFc=0
      settings: AttributesFormatString=|
      | %<ID>
      | %<Vbase>V
      | %<VLF>pu
      | %<angleLF>deg.
      | %<Name>
  bus18 : powerlib/Measurements/Load Flow Bus  LConnTagsString=a  Phases=single  Connectors=on one side  ID=bus18  Vbase=132000  Vref=1  Vangle=0  VLF=1  VLFb=1  VLFc=1  angleLF=0  angleLFb=0  angleLFc=0
      settings: AttributesFormatString=|
      | %<ID>
      | %<Vbase>V
      | %<VLF>pu
      | %<angleLF>deg.
      | %<Name>
  bus180 : powerlib/Measurements/Load Flow Bus  LConnTagsString=a  Phases=single  Connectors=on one side  ID=bus180  Vbase=400000  Vref=1  Vangle=0  VLF=1  VLFb=1  VLFc=1  angleLF=0  angleLFb=0  angleLFc=0
      settings: AttributesFormatString=|
      | %<ID>
      | %<Vbase>V
      | %<VLF>pu
      | %<angleLF>deg.
      | %<Name>
  bus181 : powerlib/Measurements/Load Flow Bus  LConnTagsString=a  Phases=single  Connectors=on one side  ID=bus181  Vbase=400000  Vref=1  Vangle=0  VLF=1  VLFb=1  VLFc=1  angleLF=0  angleLFb=0  angleLFc=0
      settings: AttributesFormatString=|
      | %<ID>
      | %<Vbase>V
      | %<VLF>pu
      | %<angleLF>deg.
      | %<Name>
  bus182 : powerlib/Measurements/Load Flow Bus  LConnTagsString=a  Phases=single  Connectors=on one side  ID=bus182  Vbase=400000  Vref=1  Vangle=0  VLF=1  VLFb=1  VLFc=1  angleLF=0  angleLFb=0  angleLFc=0
      settings: AttributesFormatString=|
      | %<ID>
      | %<Vbase>V
      | %<VLF>pu
      | %<angleLF>deg.
      | %<Name>
  bus183 : powerlib/Measurements/Load Flow Bus  LConnTagsString=a  Phases=single  Connectors=on one side  ID=bus183  Vbase=400000  Vref=1  Vangle=0  VLF=1  VLFb=1  VLFc=1  angleLF=0  angleLFb=0  angleLFc=0
      settings: AttributesFormatString=|
      | %<ID>
      | %<Vbase>V
      | %<VLF>pu
      | %<angleLF>deg.
      | %<Name>
  bus184 : powerlib/Measurements/Load Flow Bus  LConnTagsString=a  Phases=single  Connectors=on one side  ID=bus184  Vbase=400000  Vref=1  Vangle=0  VLF=1  VLFb=1  VLFc=1  angleLF=0  angleLFb=0  angleLFc=0
      settings: AttributesFormatString=|
      | %<ID>
      | %<Vbase>V
      | %<VLF>pu
      | %<angleLF>deg.
      | %<Name>
  bus185 : powerlib/Measurements/Load Flow Bus  LConnTagsString=a  Phases=single  Connectors=on one side  ID=bus185  Vbase=400000  Vref=1  Vangle=0  VLF=1  VLFb=1  VLFc=1  angleLF=0  angleLFb=0  angleLFc=0
      settings: AttributesFormatString=|
      | %<ID>
      | %<Vbase>V
      | %<VLF>pu
      | %<angleLF>deg.
      | %<Name>
  bus186 : powerlib/Measurements/Load Flow Bus  LConnTagsString=a  Phases=single  Connectors=on one side  ID=bus186  Vbase=400000  Vref=1  Vangle=0  VLF=1  VLFb=1  VLFc=1  angleLF=0  angleLFb=0  angleLFc=0
      settings: AttributesFormatString=|
      | %<ID>
      | %<Vbase>V
      | %<VLF>pu
      | %<angleLF>deg.
      | %<Name>
  bus187 : powerlib/Measurements/Load Flow Bus  LConnTagsString=a  Phases=single  Connectors=on one side  ID=bus187  Vbase=400000  Vref=1  Vangle=0  VLF=1  VLFb=1  VLFc=1  angleLF=0  angleLFb=0  angleLFc=0
      settings: AttributesFormatString=|
      | %<ID>
      | %<Vbase>V
      | %<VLF>pu
      | %<angleLF>deg.
      | %<Name>
  bus188 : powerlib/Measurements/Load Flow Bus  LConnTagsString=a  Phases=single  Connectors=on one side  ID=bus188  Vbase=400000  Vref=1  Vangle=0  VLF=1  VLFb=1  VLFc=1  angleLF=0  angleLFb=0  angleLFc=0
      settings: AttributesFormatString=|
      | %<ID>
      | %<Vbase>V
      | %<VLF>pu
      | %<angleLF>deg.
      | %<Name>
  bus189 : powerlib/Measurements/Load Flow Bus  LConnTagsString=a  Phases=single  Connectors=on one side  ID=bus189  Vbase=400000  Vref=1  Vangle=0  VLF=1  VLFb=1  VLFc=1  angleLF=0  angleLFb=0  angleLFc=0
      settings: AttributesFormatString=|
      | %<ID>
      | %<Vbase>V
      | %<VLF>pu
      | %<angleLF>deg.
      | %<Name>
  bus19 : powerlib/Measurements/Load Flow Bus  LConnTagsString=a  Phases=single  Connectors=on one side  ID=bus19  Vbase=132000  Vref=1  Vangle=0  VLF=1  VLFb=1  VLFc=1  angleLF=0  angleLFb=0  angleLFc=0
      settings: AttributesFormatString=|
      | %<ID>
      | %<Vbase>V
      | %<VLF>pu
      | %<angleLF>deg.
      | %<Name>
  bus190 : powerlib/Measurements/Load Flow Bus  LConnTagsString=a  Phases=single  Connectors=on one side  ID=bus190  Vbase=400000  Vref=1  Vangle=0  VLF=1  VLFb=1  VLFc=1  angleLF=0  angleLFb=0  angleLFc=0
      settings: AttributesFormatString=|
      | %<ID>
      | %<Vbase>V
      | %<VLF>pu
      | %<angleLF>deg.
      | %<Name>
  bus191 : powerlib/Measurements/Load Flow Bus  LConnTagsString=a  Phases=single  Connectors=on one side  ID=bus191  Vbase=400000  Vref=1  Vangle=0  VLF=1  VLFb=1  VLFc=1  angleLF=0  angleLFb=0  angleLFc=0
      settings: AttributesFormatString=|
      | %<ID>
      | %<Vbase>V
      | %<VLF>pu
      | %<angleLF>deg.
      | %<Name>
  bus192 : powerlib/Measurements/Load Flow Bus  LConnTagsString=a  Phases=single  Connectors=on one side  ID=bus192  Vbase=400000  Vref=1  Vangle=0  VLF=1  VLFb=1  VLFc=1  angleLF=0  angleLFb=0  angleLFc=0
      settings: AttributesFormatString=|
      | %<ID>
      | %<Vbase>V
      | %<VLF>pu
      | %<angleLF>deg.
      | %<Name>
  bus193 : powerlib/Measurements/Load Flow Bus  LConnTagsString=a  Phases=single  Connectors=on one side  ID=bus193  Vbase=400000  Vref=1  Vangle=0  VLF=1  VLFb=1  VLFc=1  angleLF=0  angleLFb=0  angleLFc=0
      settings: AttributesFormatString=|
      | %<ID>
      | %<Vbase>V
      | %<VLF>pu
      | %<angleLF>deg.
      | %<Name>
  bus194 : powerlib/Measurements/Load Flow Bus  LConnTagsString=a  Phases=single  Connectors=on one side  ID=bus194  Vbase=400000  Vref=1  Vangle=0  VLF=1  VLFb=1  VLFc=1  angleLF=0  angleLFb=0  angleLFc=0
      settings: AttributesFormatString=|
      | %<ID>
      | %<Vbase>V
      | %<VLF>pu
      | %<angleLF>deg.
      | %<Name>
  bus195 : powerlib/Measurements/Load Flow Bus  LConnTagsString=a  Phases=single  Connectors=on one side  ID=bus195  Vbase=400000  Vref=1  Vangle=0  VLF=1  VLFb=1  VLFc=1  angleLF=0  angleLFb=0  angleLFc=0
      settings: AttributesFormatString=|
      | %<ID>
      | %<Vbase>V
      | %<VLF>pu
      | %<angleLF>deg.
      | %<Name>
  bus196 : powerlib/Measurements/Load Flow Bus  LConnTagsString=a  Phases=single  Connectors=on one side  ID=bus196  Vbase=400000  Vref=1  Vangle=0  VLF=1  VLFb=1  VLFc=1  angleLF=0  angleLFb=0  angleLFc=0
      settings: AttributesFormatString=|
      | %<ID>
      | %<Vbase>V
      | %<VLF>pu
      | %<angleLF>deg.
      | %<Name>
  bus197 : powerlib/Measurements/Load Flow Bus  LConnTagsString=a  Phases=single  Connectors=on one side  ID=bus197  Vbase=400000  Vref=1  Vangle=0  VLF=1  VLFb=1  VLFc=1  angleLF=0  angleLFb=0  angleLFc=0
      settings: AttributesFormatString=|
      | %<ID>
      | %<Vbase>V
      | %<VLF>pu
      | %<angleLF>deg.
      | %<Name>
  bus198 : powerlib/Measurements/Load Flow Bus  LConnTagsString=a  Phases=single  Connectors=on one side  ID=bus198  Vbase=400000  Vref=1  Vangle=0  VLF=1  VLFb=1  VLFc=1  angleLF=0  angleLFb=0  angleLFc=0
      settings: AttributesFormatString=|
      | %<ID>
      | %<Vbase>V
      | %<VLF>pu
      | %<angleLF>deg.
      | %<Name>
  bus199 : powerlib/Measurements/Load Flow Bus  LConnTagsString=a  Phases=single  Connectors=on one side  ID=bus199  Vbase=400000  Vref=1  Vangle=0  VLF=1  VLFb=1  VLFc=1  angleLF=0  angleLFb=0  angleLFc=0
      settings: AttributesFormatString=|
      | %<ID>
      | %<Vbase>V
      | %<VLF>pu
      | %<angleLF>deg.
      | %<Name>
  bus2 : powerlib/Measurements/Load Flow Bus  LConnTagsString=a  Phases=single  Connectors=on one side  ID=bus2  Vbase=132000  Vref=1  Vangle=0  VLF=1  VLFb=1  VLFc=1  angleLF=0  angleLFb=0  angleLFc=0
      settings: AttributesFormatString=|
      | %<ID>
      | %<Vbase>V
      | %<VLF>pu
      | %<angleLF>deg.
      | %<Name>
  bus20 : powerlib/Measurements/Load Flow Bus  LConnTagsString=a  Phases=single  Connectors=on one side  ID=bus20  Vbase=132000  Vref=1  Vangle=0  VLF=1  VLFb=1  VLFc=1  angleLF=0  angleLFb=0  angleLFc=0
      settings: AttributesFormatString=|
      | %<ID>
      | %<Vbase>V
      | %<VLF>pu
      | %<angleLF>deg.
      | %<Name>
  bus200 : powerlib/Measurements/Load Flow Bus  LConnTagsString=a  Phases=single  Connectors=on one side  ID=bus200  Vbase=400000  Vref=1  Vangle=0  VLF=1  VLFb=1  VLFc=1  angleLF=0  angleLFb=0  angleLFc=0
      settings: AttributesFormatString=|
      | %<ID>
      | %<Vbase>V
      | %<VLF>pu
      | %<angleLF>deg.
      | %<Name>
  bus201 : powerlib/Measurements/Load Flow Bus  LConnTagsString=a  Phases=single  Connectors=on one side  ID=bus201  Vbase=400000  Vref=1  Vangle=0  VLF=1  VLFb=1  VLFc=1  angleLF=0  angleLFb=0  angleLFc=0
      settings: AttributesFormatString=|
      | %<ID>
      | %<Vbase>V
      | %<VLF>pu
      | %<angleLF>deg.
      | %<Name>
  bus202 : powerlib/Measurements/Load Flow Bus  LConnTagsString=a  Phases=single  Connectors=on one side  ID=bus202  Vbase=400000  Vref=1  Vangle=0  VLF=1  VLFb=1  VLFc=1  angleLF=0  angleLFb=0  angleLFc=0
      settings: AttributesFormatString=|
      | %<ID>
      | %<Vbase>V
      | %<VLF>pu
      | %<angleLF>deg.
      | %<Name>
  bus203 : powerlib/Measurements/Load Flow Bus  LConnTagsString=a  Phases=single  Connectors=on one side  ID=bus203  Vbase=400000  Vref=1  Vangle=0  VLF=1  VLFb=1  VLFc=1  angleLF=0  angleLFb=0  angleLFc=0
      settings: AttributesFormatString=|
      | %<ID>
      | %<Vbase>V
      | %<VLF>pu
      | %<angleLF>deg.
      | %<Name>
  bus204 : powerlib/Measurements/Load Flow Bus  LConnTagsString=a  Phases=single  Connectors=on one side  ID=bus204  Vbase=400000  Vref=1  Vangle=0  VLF=1  VLFb=1  VLFc=1  angleLF=0  angleLFb=0  angleLFc=0
      settings: AttributesFormatString=|
      | %<ID>
      | %<Vbase>V
      | %<VLF>pu
      | %<angleLF>deg.
      | %<Name>
  bus205 : powerlib/Measurements/Load Flow Bus  LConnTagsString=a  Phases=single  Connectors=on one side  ID=bus205  Vbase=400000  Vref=1  Vangle=0  VLF=1  VLFb=1  VLFc=1  angleLF=0  angleLFb=0  angleLFc=0
      settings: AttributesFormatString=|
      | %<ID>
      | %<Vbase>V
      | %<VLF>pu
      | %<angleLF>deg.
      | %<Name>
  bus206 : powerlib/Measurements/Load Flow Bus  LConnTagsString=a  Phases=single  Connectors=on one side  ID=bus206  Vbase=400000  Vref=1  Vangle=0  VLF=1  VLFb=1  VLFc=1  angleLF=0  angleLFb=0  angleLFc=0
      settings: AttributesFormatString=|
      | %<ID>
      | %<Vbase>V
      | %<VLF>pu
      | %<angleLF>deg.
      | %<Name>
  bus207 : powerlib/Measurements/Load Flow Bus  LConnTagsString=a  Phases=single  Connectors=on one side  ID=bus207  Vbase=400000  Vref=1  Vangle=0  VLF=1  VLFb=1  VLFc=1  angleLF=0  angleLFb=0  angleLFc=0
      settings: AttributesFormatString=|
      | %<ID>
      | %<Vbase>V
      | %<VLF>pu
      | %<angleLF>deg.
      | %<Name>
  bus208 : powerlib/Measurements/Load Flow Bus  LConnTagsString=a  Phases=single  Connectors=on one side  ID=bus208  Vbase=400000  Vref=1  Vangle=0  VLF=1  VLFb=1  VLFc=1  angleLF=0  angleLFb=0  angleLFc=0
      settings: AttributesFormatString=|
      | %<ID>
      | %<Vbase>V
      | %<VLF>pu
      | %<angleLF>deg.
      | %<Name>
  bus209 : powerlib/Measurements/Load Flow Bus  LConnTagsString=a  Phases=single  Connectors=on one side  ID=bus209  Vbase=400000  Vref=1  Vangle=0  VLF=1  VLFb=1  VLFc=1  angleLF=0  angleLFb=0  angleLFc=0
      settings: AttributesFormatString=|
      | %<ID>
      | %<Vbase>V
      | %<VLF>pu
      | %<angleLF>deg.
      | %<Name>
  bus21 : powerlib/Measurements/Load Flow Bus  LConnTagsString=a  Phases=single  Connectors=on one side  ID=bus21  Vbase=132000  Vref=1  Vangle=0  VLF=1  VLFb=1  VLFc=1  angleLF=0  angleLFb=0  angleLFc=0
      settings: AttributesFormatString=|
      | %<ID>
      | %<Vbase>V
      | %<VLF>pu
      | %<angleLF>deg.
      | %<Name>
  bus210 : powerlib/Measurements/Load Flow Bus  LConnTagsString=a  Phases=single  Connectors=on one side  ID=bus210  Vbase=400000  Vref=1  Vangle=0  VLF=1  VLFb=1  VLFc=1  angleLF=0  angleLFb=0  angleLFc=0
      settings: AttributesFormatString=|
      | %<ID>
      | %<Vbase>V
      | %<VLF>pu
      | %<angleLF>deg.
      | %<Name>
  bus211 : powerlib/Measurements/Load Flow Bus  LConnTagsString=a  Phases=single  Connectors=on one side  ID=bus211  Vbase=400000  Vref=1  Vangle=0  VLF=1  VLFb=1  VLFc=1  angleLF=0  angleLFb=0  angleLFc=0
      settings: AttributesFormatString=|
      | %<ID>
      | %<Vbase>V
      | %<VLF>pu
      | %<angleLF>deg.
      | %<Name>
  bus212 : powerlib/Measurements/Load Flow Bus  LConnTagsString=a  Phases=single  Connectors=on one side  ID=bus212  Vbase=400000  Vref=1  Vangle=0  VLF=1  VLFb=1  VLFc=1  angleLF=0  angleLFb=0  angleLFc=0
      settings: AttributesFormatString=|
      | %<ID>
      | %<Vbase>V
      | %<VLF>pu
      | %<angleLF>deg.
      | %<Name>
  bus213 : powerlib/Measurements/Load Flow Bus  LConnTagsString=a  Phases=single  Connectors=on one side  ID=bus213  Vbase=400000  Vref=1  Vangle=0  VLF=1  VLFb=1  VLFc=1  angleLF=0  angleLFb=0  angleLFc=0
